simulink library "outp"  (R2021b)
(part 5 of 8)

  VBCM_MirrorFlodPos_flg_Inproc : FVT_lib/outp/OverrideAndLimit  SystemSampleTime=-1  VariantActivationTime=update diagram  Latency=0  AutoFrameSizeCalculation=off
      link override Signal_Limit/_maxval: Value=KOUTP_MirrorFlodPos_flg_maxval
      link override Signal_Limit/_minval: Value=KOUTP_MirrorFlodPos_flg_minval
      link override Signal_Override/_ovrdflg: Value=KOUTP_MirrorFlodPos_flg_ovrdflg
      link override Signal_Override/_ovrdval: Value=KOUTP_MirrorFlodPos_flg_ovrdval
  VBCM_OutMode_enum_Inproc : FVT_lib/outp/OverrideAndLimit  SystemSampleTime=-1  VariantActivationTime=update diagram  Latency=0  AutoFrameSizeCalculation=off
      link override Signal_Limit/_maxval: Value=KOUTP_OutMode_enum_maxval
      link override Signal_Limit/_minval: Value=KOUTP_OutMode_enum_minval
      link override Signal_Override/_ovrdflg: Value=KOUTP_OutMode_enum_ovrdflg
      link override Signal_Override/_ovrdval: Value=KOUTP_OutMode_enum_ovrdval
  VBCM_PTGInnerSW2_enum_Inproc : FVT_lib/outp/OverrideAndLimit  SystemSampleTime=-1  VariantActivationTime=update diagram  Latency=0  AutoFrameSizeCalculation=off
      link override Signal_Limit/_maxval: Value=KOUTP_PTGInnerSW2_enum_maxval
      link override Signal_Limit/_minval: Value=KOUTP_PTGInnerSW2_enum_minval
      link override Signal_Override/_ovrdflg: Value=KOUTP_PTGInnerSW2_enum_ovrdflg
      link override Signal_Override/_ovrdval: Value=KOUTP_PTGInnerSW2_enum_ovrdval
  VBCM_PosLamp_flg_Inproc : FVT_lib/outp/OverrideAndLimit  SystemSampleTime=-1  VariantActivationTime=update diagram  Latency=0  AutoFrameSizeCalculation=off
      link override Signal_Limit/_maxval: Value=KOUTP_PosLamp_flg_maxval
      link override Signal_Limit/_minval: Value=KOUTP_PosLamp_flg_minval
      link override Signal_Override/_ovrdflg: Value=KOUTP_PosLamp_flg_ovrdflg
      link override Signal_Override/_ovrdval: Value=KOUTP_PosLamp_flg_ovrdval
  VBCM_PsDoorSW_flg_Inproc : FVT_lib/outp/OverrideAndLimit  SystemSampleTime=-1  VariantActivationTime=update diagram  Latency=0  AutoFrameSizeCalculation=off
      link override Signal_Limit/_maxval: Value=KOUTP_PsDoorSW_flg_maxval
      link override Signal_Limit/_minval: Value=KOUTP_PsDoorSW_flg_minval
      link override Signal_Override/_ovrdflg: Value=KOUTP_PsDoorSW_flg_ovrdflg
      link override Signal_Override/_ovrdval: Value=KOUTP_PsDoorSW_flg_ovrdval
  VBCM_RBSD_flg_Inproc : FVT_lib/outp/OverrideAndLimit  SystemSampleTime=-1  VariantActivationTime=update diagram  Latency=0  AutoFrameSizeCalculation=off
      link override Signal_Limit/_maxval: Value=KOUTP_RBSD_flg_maxval
      link override Signal_Limit/_minval: Value=KOUTP_RBSD_flg_minval
      link override Signal_Override/_ovrdflg: Value=KOUTP_RBSD_flg_ovrdflg
      link override Signal_Override/_ovrdval: Value=KOUTP_RBSD_flg_ovrdval
  VBCM_RDRL_flg_Inproc : FVT_lib/outp/OverrideAndLimit  SystemSampleTime=-1  VariantActivationTime=update diagram  Latency=0  AutoFrameSizeCalculation=off
      link override Signal_Limit/_maxval: Value=KOUTP_RDRL_flg_maxval
      link override Signal_Limit/_minval: Value=KOUTP_RDRL_flg_minval
      link override Signal_Override/_ovrdflg: Value=KOUTP_RDRL_flg_ovrdflg
      link override Signal_Override/_ovrdval: Value=KOUTP_RDRL_flg_ovrdval
  VBCM_RLDoorSW_flg_Inproc : FVT_lib/outp/OverrideAndLimit  SystemSampleTime=-1  VariantActivationTime=update diagram  Latency=0  AutoFrameSizeCalculation=off
      link override Signal_Limit/_maxval: Value=KOUTP_RLDoorSW_flg_maxval
      link override Signal_Limit/_minval: Value=KOUTP_RLDoorSW_flg_minval
      link override Signal_Override/_ovrdflg: Value=KOUTP_RLDoorSW_flg_ovrdflg
      link override Signal_Override/_ovrdval: Value=KOUTP_RLDoorSW_flg_ovrdval
  VBCM_RRDoorSW_flg_Inproc : FVT_lib/outp/OverrideAndLimit  SystemSampleTime=-1  VariantActivationTime=update diagram  Latency=0  AutoFrameSizeCalculation=off
      link override Signal_Limit/_maxval: Value=KOUTP_RRDoorSW_flg_maxval
      link override Signal_Limit/_minval: Value=KOUTP_RRDoorSW_flg_minval
      link override Signal_Override/_ovrdflg: Value=KOUTP_RRDoorSW_flg_ovrdflg
      link override Signal_Override/_ovrdval: Value=KOUTP_RRDoorSW_flg_ovrdval
  VBCM_RTurnLP_flg_Inproc : FVT_lib/outp/OverrideAndLimit  SystemSampleTime=-1  VariantActivationTime=update diagram  Latency=0  AutoFrameSizeCalculation=off
      link override Signal_Limit/_maxval: Value=KOUTP_RTurnLP_flg_maxval
      link override Signal_Limit/_minval: Value=KOUTP_RTurnLP_flg_minval
      link override Signal_Override/_ovrdflg: Value=KOUTP_RTurnLP_flg_ovrdflg
      link override Signal_Override/_ovrdval: Value=KOUTP_RTurnLP_flg_ovrdval
  VBCM_ReverseLamp_flg_Inproc : FVT_lib/outp/OverrideAndLimit  SystemSampleTime=-1  VariantActivationTime=update diagram  Latency=0  AutoFrameSizeCalculation=off
      link override Signal_Limit/_maxval: Value=KOUTP_ReverseLamp_flg_maxval
      link override Signal_Limit/_minval: Value=KOUTP_ReverseLamp_flg_minval
      link override Signal_Override/_ovrdflg: Value=KOUTP_ReverseLamp_flg_ovrdflg
      link override Signal_Override/_ovrdval: Value=KOUTP_ReverseLamp_flg_ovrdval
  VBCM_RoomLampH_flg_Inproc : FVT_lib/outp/OverrideAndLimit  SystemSampleTime=-1  VariantActivationTime=update diagram  Latency=0  AutoFrameSizeCalculation=off
      link override Signal_Limit/_maxval: Value=KOUTP_RoomLampH_flg_maxval
      link override Signal_Limit/_minval: Value=KOUTP_RoomLampH_flg_minval
      link override Signal_Override/_ovrdflg: Value=KOUTP_RoomLampH_flg_ovrdflg
      link override Signal_Override/_ovrdval: Value=KOUTP_RoomLampH_flg_ovrdval
  VBCM_RoomLampL_flg_Inproc : FVT_lib/outp/OverrideAndLimit  SystemSampleTime=-1  VariantActivationTime=update diagram  Latency=0  AutoFrameSizeCalculation=off
      link override Signal_Limit/_maxval: Value=KOUTP_RoomLampL_flg_maxval
      link override Signal_Limit/_minval: Value=KOUTP_RoomLampL_flg_minval
      link override Signal_Override/_ovrdflg: Value=KOUTP_RoomLampL_flg_ovrdflg
      link override Signal_Override/_ovrdval: Value=KOUTP_RoomLampL_flg_ovrdval
  VBCM_RoomLampMode_flg_Inproc : FVT_lib/outp/OverrideAndLimit  SystemSampleTime=-1  VariantActivationTime=update diagram  Latency=0  AutoFrameSizeCalculation=off
      link override Signal_Limit/_maxval: Value=KOUTP_RoomLampMode_flg_maxval
      link override Signal_Limit/_minval: Value=KOUTP_RoomLampMode_flg_minval
      link override Signal_Override/_ovrdflg: Value=KOUTP_RoomLampMode_flg_ovrdflg
      link override Signal_Override/_ovrdval: Value=KOUTP_RoomLampMode_flg_ovrdval
  VBCM_RrChargingDoorCtrl_enum_Inproc : FVT_lib/outp/OverrideAndLimit  SystemSampleTime=-1  VariantActivationTime=update diagram  Latency=0  AutoFrameSizeCalculation=off
      link override Signal_Limit/_maxval: Value=KOUTP_RrChargingDoorCtrl_enum_maxval
      link override Signal_Limit/_minval: Value=KOUTP_RrChargingDoorCtrl_enum_minval
      link override Signal_Override/_ovrdflg: Value=KOUTP_RrChargingDoorCtrl_enum_ovrdflg
      link override Signal_Override/_ovrdval: Value=KOUTP_RrChargingDoorCtrl_enum_ovrdval
  VBCM_RrDefog_flg_Inproc : FVT_lib/outp/OverrideAndLimit  SystemSampleTime=-1  VariantActivationTime=update diagram  Latency=0  AutoFrameSizeCalculation=off
      link override Signal_Limit/_maxval: Value=KOUTP_RrDefog_flg_maxval
      link override Signal_Limit/_minval: Value=KOUTP_RrDefog_flg_minval
      link override Signal_Override/_ovrdflg: Value=KOUTP_RrDefog_flg_ovrdflg
      link override Signal_Override/_ovrdval: Value=KOUTP_RrDefog_flg_ovrdval
  VBCM_RrFogLamp_flg_Inproc : FVT_lib/outp/OverrideAndLimit  SystemSampleTime=-1  VariantActivationTime=update diagram  Latency=0  AutoFrameSizeCalculation=off
      link override Signal_Limit/_maxval: Value=KOUTP_RrFogLamp_flg_maxval
      link override Signal_Limit/_minval: Value=KOUTP_RrFogLamp_flg_minval
      link override Signal_Override/_ovrdflg: Value=KOUTP_RrFogLamp_flg_ovrdflg
      link override Signal_Override/_ovrdval: Value=KOUTP_RrFogLamp_flg_ovrdval
  VBCM_RrWiper_flg_Inproc : FVT_lib/outp/OverrideAndLimit  SystemSampleTime=-1  VariantActivationTime=update diagram  Latency=0  AutoFrameSizeCalculation=off
      link override Signal_Limit/_maxval: Value=KOUTP_RrWiper_flg_maxval
      link override Signal_Limit/_minval: Value=KOUTP_RrWiper_flg_minval
      link override Signal_Override/_ovrdflg: Value=KOUTP_RrWiper_flg_ovrdflg
      link override Signal_Override/_ovrdval: Value=KOUTP_RrWiper_flg_ovrdval
  VBCM_SPTGDet_flg_Inproc : FVT_lib/outp/OverrideAndLimit  SystemSampleTime=-1  VariantActivationTime=update diagram  Latency=0  AutoFrameSizeCalculation=off
      link override Signal_Limit/_maxval: Value=KOUTP_SPTGDet_flg_maxval
      link override Signal_Limit/_minval: Value=KOUTP_SPTGDet_flg_minval
      link override Signal_Override/_ovrdflg: Value=KOUTP_SPTGDet_flg_ovrdflg
      link override Signal_Override/_ovrdval: Value=KOUTP_SPTGDet_flg_ovrdval
  VBCM_TailgateHDSW_flg_Inproc : FVT_lib/outp/OverrideAndLimit  SystemSampleTime=-1  VariantActivationTime=update diagram  Latency=0  AutoFrameSizeCalculation=off
      link override Signal_Limit/_maxval: Value=KOUTP_TailgateHDSW_flg_maxval
      link override Signal_Limit/_minval: Value=KOUTP_TailgateHDSW_flg_minval
      link override Signal_Override/_ovrdflg: Value=KOUTP_TailgateHDSW_flg_ovrdflg
      link override Signal_Override/_ovrdval: Value=KOUTP_TailgateHDSW_flg_ovrdval
  VBCM_TailgateRemote_enum_Inproc : FVT_lib/outp/OverrideAndLimit  SystemSampleTime=-1  VariantActivationTime=update diagram  Latency=0  AutoFrameSizeCalculation=off
      link override Signal_Limit/_maxval: Value=KOUTP_TailgateRemote_enum_maxval
      link override Signal_Limit/_minval: Value=KOUTP_TailgateRemote_enum_minval
      link override Signal_Override/_ovrdflg: Value=KOUTP_TailgateRemote_enum_ovrdflg
      link override Signal_Override/_ovrdval: Value=KOUTP_TailgateRemote_enum_ovrdval
  VBCM_TailgateSW_flg_Inproc : FVT_lib/outp/OverrideAndLimit  SystemSampleTime=-1  VariantActivationTime=update diagram  Latency=0  AutoFrameSizeCalculation=off
      link override Signal_Limit/_maxval: Value=KOUTP_TailgateSW_flg_maxval
      link override Signal_Limit/_minval: Value=KOUTP_TailgateSW_flg_minval
      link override Signal_Override/_ovrdflg: Value=KOUTP_TailgateSW_flg_ovrdflg
      link override Signal_Override/_ovrdval: Value=KOUTP_TailgateSW_flg_ovrdval
  VBCM_TrunkRel_flg_Inproc : FVT_lib/outp/OverrideAndLimit  SystemSampleTime=-1  VariantActivationTime=update diagram  Latency=0  AutoFrameSizeCalculation=off
      link override Signal_Limit/_maxval: Value=KOUTP_TrunkRel_flg_maxval
      link override Signal_Limit/_minval: Value=KOUTP_TrunkRel_flg_minval
      link override Signal_Override/_ovrdflg: Value=KOUTP_TrunkRel_flg_ovrdflg
      link override Signal_Override/_ovrdval: Value=KOUTP_TrunkRel_flg_ovrdval
  VBCM_User1AmbLightColor_enum_Inproc : FVT_lib/outp/OverrideAndLimit  SystemSampleTime=-1  VariantActivationTime=update diagram  Latency=0  AutoFrameSizeCalculation=off
      link override Signal_Limit/_maxval: Value=KOUTP_User1AmbLightColor_enum_maxval
      link override Signal_Limit/_minval: Value=KOUTP_User1AmbLightColor_enum_minval
      link override Signal_Override/_ovrdflg: Value=KOUTP_User1AmbLightColor_enum_ovrdflg
      link override Signal_Override/_ovrdval: Value=KOUTP_User1AmbLightColor_enum_ovrdval
  VBCM_User1DrAmbLightBrightness_enum_Inproc : FVT_lib/outp/OverrideAndLimit  SystemSampleTime=-1  VariantActivationTime=update diagram  Latency=0  AutoFrameSizeCalculation=off
      link override Signal_Limit/_maxval: Value=KOUTP_User1DrAmbLightBrightness_enum_maxval
      link override Signal_Limit/_minval: Value=KOUTP_User1DrAmbLightBrightness_enum_minval
      link override Signal_Override/_ovrdflg: Value=KOUTP_User1DrAmbLightBrightness_enum_ovrdflg
      link override Signal_Override/_ovrdval: Value=KOUTP_User1DrAmbLightBrightness_enum_ovrdval
  VBCM_User1IPAmbLightBrightness_enum_Inproc : FVT_lib/outp/OverrideAndLimit  SystemSampleTime=-1  VariantActivationTime=update diagram  Latency=0  AutoFrameSizeCalculation=off
      link override Signal_Limit/_maxval: Value=KOUTP_User1IPAmbLightBrightness_enum_maxval
      link override Signal_Limit/_minval: Value=KOUTP_User1IPAmbLightBrightness_enum_minval
      link override Signal_Override/_ovrdflg: Value=KOUTP_User1IPAmbLightBrightness_enum_ovrdflg
      link override Signal_Override/_ovrdval: Value=KOUTP_User1IPAmbLightBrightness_enum_ovrdval
  VBCM_User2AmbLightColor_enum_Inproc : FVT_lib/outp/OverrideAndLimit  SystemSampleTime=-1  VariantActivationTime=update diagram  Latency=0  AutoFrameSizeCalculation=off
      link override Signal_Limit/_maxval: Value=KOUTP_User2AmbLightColor_enum_maxval
      link override Signal_Limit/_minval: Value=KOUTP_User2AmbLightColor_enum_minval
      link override Signal_Override/_ovrdflg: Value=KOUTP_User2AmbLightColor_enum_ovrdflg
      link override Signal_Override/_ovrdval: Value=KOUTP_User2AmbLightColor_enum_ovrdval
  VBCM_User2DrAmbLightBrightness_enum_Inproc : FVT_lib/outp/OverrideAndLimit  SystemSampleTime=-1  VariantActivationTime=update diagram  Latency=0  AutoFrameSizeCalculation=off
      link override Signal_Limit/_maxval: Value=KOUTP_User2DrAmbLightBrightness_enum_maxval
      link override Signal_Limit/_minval: Value=KOUTP_User2DrAmbLightBrightness_enum_minval
      link override Signal_Override/_ovrdflg: Value=KOUTP_User2DrAmbLightBrightness_enum_ovrdflg
      link override Signal_Override/_ovrdval: Value=KOUTP_User2DrAmbLightBrightness_enum_ovrdval
  VBCM_User2IPAmbLightBrightness_enum_Inproc : FVT_lib/outp/OverrideAndLimit  SystemSampleTime=-1  VariantActivationTime=update diagram  Latency=0  AutoFrameSizeCalculation=off
      link override Signal_Limit/_maxval: Value=KOUTP_User2IPAmbLightBrightness_enum_maxval
      link override Signal_Limit/_minval: Value=KOUTP_User2IPAmbLightBrightness_enum_minval
      link override Signal_Override/_ovrdflg: Value=KOUTP_User2IPAmbLightBrightness_enum_ovrdflg
      link override Signal_Override/_ovrdval: Value=KOUTP_User2IPAmbLightBrightness_enum_ovrdval
  VBCM_User3AmbLightColor_enum_Inproc : FVT_lib/outp/OverrideAndLimit  SystemSampleTime=-1  VariantActivationTime=update diagram  Latency=0  AutoFrameSizeCalculation=off
      link override Signal_Limit/_maxval: Value=KOUTP_User3AmbLightColor_enum_maxval
      link override Signal_Limit/_minval: Value=KOUTP_User3AmbLightColor_enum_minval
      link override Signal_Override/_ovrdflg: Value=KOUTP_User3AmbLightColor_enum_ovrdflg
      link override Signal_Override/_ovrdval: Value=KOUTP_User3AmbLightColor_enum_ovrdval
  VBCM_User3DrAmbLightBrightness_enum_Inproc : FVT_lib/outp/OverrideAndLimit  SystemSampleTime=-1  VariantActivationTime=update diagram  Latency=0  AutoFrameSizeCalculation=off
      link override Signal_Limit/_maxval: Value=KOUTP_User3DrAmbLightBrightness_enum_maxval
      link override Signal_Limit/_minval: Value=KOUTP_User3DrAmbLightBrightness_enum_minval
      link override Signal_Override/_ovrdflg: Value=KOUTP_User3DrAmbLightBrightness_enum_ovrdflg
      link override Signal_Override/_ovrdval: Value=KOUTP_User3DrAmbLightBrightness_enum_ovrdval
  VBCM_User3IPAmbLightBrightness_enum_Inproc : FVT_lib/outp/OverrideAndLimit  SystemSampleTime=-1  VariantActivationTime=update diagram  Latency=0  AutoFrameSizeCalculation=off
      link override Signal_Limit/_maxval: Value=KOUTP_User3IPAmbLightBrightness_enum_maxval
      link override Signal_Limit/_minval: Value=KOUTP_User3IPAmbLightBrightness_enum_minval
      link override Signal_Override/_ovrdflg: Value=KOUTP_User3IPAmbLightBrightness_enum_ovrdflg
      link override Signal_Override/_ovrdval: Value=KOUTP_User3IPAmbLightBrightness_enum_ovrdval
  VBCM_User4AmbLightColor_enum_Inproc : FVT_lib/outp/OverrideAndLimit  SystemSampleTime=-1  VariantActivationTime=update diagram  Latency=0  AutoFrameSizeCalculation=off
      link override Signal_Limit/_maxval: Value=KOUTP_User4AmbLightColor_enum_maxval
      link override Signal_Limit/_minval: Value=KOUTP_User4AmbLightColor_enum_minval
      link override Signal_Override/_ovrdflg: Value=KOUTP_User4AmbLightColor_enum_ovrdflg
      link override Signal_Override/_ovrdval: Value=KOUTP_User4AmbLightColor_enum_ovrdval
  VBCM_User4DrAmbLightBrightness_enum_Inproc : FVT_lib/outp/OverrideAndLimit  SystemSampleTime=-1  VariantActivationTime=update diagram  Latency=0  AutoFrameSizeCalculation=off
      link override Signal_Limit/_maxval: Value=KOUTP_User4DrAmbLightBrightness_enum_maxval
      link override Signal_Limit/_minval: Value=KOUTP_User4DrAmbLightBrightness_enum_minval
      link override Signal_Override/_ovrdflg: Value=KOUTP_User4DrAmbLightBrightness_enum_ovrdflg
      link override Signal_Override/_ovrdval: Value=KOUTP_User4DrAmbLightBrightness_enum_ovrdval
  VBCM_User4IPAmbLightBrightness_enum_Inproc : FVT_lib/outp/OverrideAndLimit  SystemSampleTime=-1  VariantActivationTime=update diagram  Latency=0  AutoFrameSizeCalculation=off
      link override Signal_Limit/_maxval: Value=KOUTP_User4IPAmbLightBrightness_enum_maxval
      link override Signal_Limit/_minval: Value=KOUTP_User4IPAmbLightBrightness_enum_minval
      link override Signal_Override/_ovrdflg: Value=KOUTP_User4IPAmbLightBrightness_enum_ovrdflg
      link override Signal_Override/_ovrdval: Value=KOUTP_User4IPAmbLightBrightness_enum_ovrdval
  VBCM_User5AmbLightColor_enum_Inproc : FVT_lib/outp/OverrideAndLimit  SystemSampleTime=-1  VariantActivationTime=update diagram  Latency=0  AutoFrameSizeCalculation=off
      link override Signal_Limit/_maxval: Value=KOUTP_User5AmbLightColor_enum_maxval
      link override Signal_Limit/_minval: Value=KOUTP_User5AmbLightColor_enum_minval
      link override Signal_Override/_ovrdflg: Value=KOUTP_User5AmbLightColor_enum_ovrdflg
      link override Signal_Override/_ovrdval: Value=KOUTP_User5AmbLightColor_enum_ovrdval
  VBCM_User5DrAmbLightBrightness_enum_Inproc : FVT_lib/outp/OverrideAndLimit  SystemSampleTime=-1  VariantActivationTime=update diagram  Latency=0  AutoFrameSizeCalculation=off
      link override Signal_Limit/_maxval: Value=KOUTP_User5DrAmbLightBrightness_enum_maxval
      link override Signal_Limit/_minval: Value=KOUTP_User5DrAmbLightBrightness_enum_minval
      link override Signal_Override/_ovrdflg: Value=KOUTP_User5DrAmbLightBrightness_enum_ovrdflg
      link override Signal_Override/_ovrdval: Value=KOUTP_User5DrAmbLightBrightness_enum_ovrdval
  VBCM_User5IPAmbLightBrightness_enum_Inproc : FVT_lib/outp/OverrideAndLimit  SystemSampleTime=-1  VariantActivationTime=update diagram  Latency=0  AutoFrameSizeCalculation=off
      link override Signal_Limit/_maxval: Value=KOUTP_User5IPAmbLightBrightness_enum_maxval
      link override Signal_Limit/_minval: Value=KOUTP_User5IPAmbLightBrightness_enum_minval
      link override Signal_Override/_ovrdflg: Value=KOUTP_User5IPAmbLightBrightness_enum_ovrdflg
      link override Signal_Override/_ovrdval: Value=KOUTP_User5IPAmbLightBrightness_enum_ovrdval
  VBCM_User6AmbLightColor_enum_Inproc : FVT_lib/outp/OverrideAndLimit  SystemSampleTime=-1  VariantActivationTime=update diagram  Latency=0  AutoFrameSizeCalculation=off
      link override Signal_Limit/_maxval: Value=KOUTP_User6AmbLightColor_enum_maxval
      link override Signal_Limit/_minval: Value=KOUTP_User6AmbLightColor_enum_minval
      link override Signal_Override/_ovrdflg: Value=KOUTP_User6AmbLightColor_enum_ovrdflg
      link override Signal_Override/_ovrdval: Value=KOUTP_User6AmbLightColor_enum_ovrdval
  VBCM_User6DrAmbLightBrightness_enum_Inproc : FVT_lib/outp/OverrideAndLimit  SystemSampleTime=-1  VariantActivationTime=update diagram  Latency=0  AutoFrameSizeCalculation=off
      link override Signal_Limit/_maxval: Value=KOUTP_User6DrAmbLightBrightness_enum_maxval
      link override Signal_Limit/_minval: Value=KOUTP_User6DrAmbLightBrightness_enum_minval
      link override Signal_Override/_ovrdflg: Value=KOUTP_User6DrAmbLightBrightness_enum_ovrdflg
      link override Signal_Override/_ovrdval: Value=KOUTP_User6DrAmbLightBrightness_enum_ovrdval
  VBCM_User6IPAmbLightBrightness_enum_Inproc : FVT_lib/outp/OverrideAndLimit  SystemSampleTime=-1  VariantActivationTime=update diagram  Latency=0  AutoFrameSizeCalculation=off
      link override Signal_Limit/_maxval: Value=KOUTP_User6IPAmbLightBrightness_enum_maxval
      link override Signal_Limit/_minval: Value=KOUTP_User6IPAmbLightBrightness_enum_minval
      link override Signal_Override/_ovrdflg: Value=KOUTP_User6IPAmbLightBrightness_enum_ovrdflg
      link override Signal_Override/_ovrdval: Value=KOUTP_User6IPAmbLightBrightness_enum_ovrdval
  VBCM_WasherCtrl_enum_Inproc : FVT_lib/outp/OverrideAndLimit  SystemSampleTime=-1  VariantActivationTime=update diagram  Latency=0  AutoFrameSizeCalculation=off
      link override Signal_Limit/_maxval: Value=KOUTP_WasherCtrl_enum_maxval
      link override Signal_Limit/_minval: Value=KOUTP_WasherCtrl_enum_minval
      link override Signal_Override/_ovrdflg: Value=KOUTP_WasherCtrl_enum_ovrdflg
      link override Signal_Override/_ovrdval: Value=KOUTP_WasherCtrl_enum_ovrdval
  VBCM_WiperFixMode_flg_Inproc : FVT_lib/outp/OverrideAndLimit  SystemSampleTime=-1  VariantActivationTime=update diagram  Latency=0  AutoFrameSizeCalculation=off
      link override Signal_Limit/_maxval: Value=KOUTP_WiperFixMode_flg_maxval
      link override Signal_Limit/_minval: Value=KOUTP_WiperFixMode_flg_minval
      link override Signal_Override/_ovrdflg: Value=KOUTP_WiperFixMode_flg_ovrdflg
      link override Signal_Override/_ovrdval: Value=KOUTP_WiperFixMode_flg_ovrdval
  VBCM_fUnlockSingle_flg_Inproc : FVT_lib/outp/OverrideAndLimit  SystemSampleTime=-1  VariantActivationTime=update diagram  Latency=0  AutoFrameSizeCalculation=off
      link override Signal_Limit/_maxval: Value=KOUTP_fUnlockSingle_flg_maxval
      link override Signal_Limit/_minval: Value=KOUTP_fUnlockSingle_flg_minval
      link override Signal_Override/_ovrdflg: Value=KOUTP_fUnlockSingle_flg_ovrdflg
      link override Signal_Override/_ovrdval: Value=KOUTP_fUnlockSingle_flg_ovrdval
  VDDM_5vAPS1PwrErrDTC_raw32_Inproc : FVT_lib/outp/OverrideAndLimit  SystemSampleTime=-1  VariantActivationTime=update diagram  Latency=0  AutoFrameSizeCalculation=off
      link override Signal_Limit/_maxval: Value=KOUTP_5vAPS1PwrErrDTC_raw32_maxval
      link override Signal_Limit/_minval: Value=KOUTP_5vAPS1PwrErrDTC_raw32_minval
      link override Signal_Override/_ovrdflg: Value=KOUTP_5vAPS1PwrErrDTC_raw32_ovrdflg
      link override Signal_Override/_ovrdval: Value=KOUTP_5vAPS1PwrErrDTC_raw32_ovrdval
  VDDM_5vAPS2PwrErrDTC_raw32_Inproc : FVT_lib/outp/OverrideAndLimit  SystemSampleTime=-1  VariantActivationTime=update diagram  Latency=0  AutoFrameSizeCalculation=off
      link override Signal_Limit/_maxval: Value=KOUTP_5vAPS2PwrErrDTC_raw32_maxval
      link override Signal_Limit/_minval: Value=KOUTP_5vAPS2PwrErrDTC_raw32_minval
      link override Signal_Override/_ovrdflg: Value=KOUTP_5vAPS2PwrErrDTC_raw32_ovrdflg
      link override Signal_Override/_ovrdval: Value=KOUTP_5vAPS2PwrErrDTC_raw32_ovrdval
  VDDM_ACCAccelCmdErrDetDTC_raw32_Inproc : FVT_lib/outp/OverrideAndLimit  SystemSampleTime=-1  VariantActivationTime=update diagram  Latency=0  AutoFrameSizeCalculation=off
      link override Signal_Limit/_maxval: Value=KOUTP_ACCAccelCmdErrDetDTC_raw32_maxval
      link override Signal_Limit/_minval: Value=KOUTP_ACCAccelCmdErrDetDTC_raw32_minval
      link override Signal_Override/_ovrdflg: Value=KOUTP_ACCAccelCmdErrDetDTC_raw32_ovrdflg
      link override Signal_Override/_ovrdval: Value=KOUTP_ACCAccelCmdErrDetDTC_raw32_ovrdval
  VDDM_ACCMalfuncDetDTC_raw32_Inproc : FVT_lib/outp/OverrideAndLimit  SystemSampleTime=-1  VariantActivationTime=update diagram  Latency=0  AutoFrameSizeCalculation=off
      link override Signal_Limit/_maxval: Value=KOUTP_ACCMalfuncDetDTC_raw32_maxval
      link override Signal_Limit/_minval: Value=KOUTP_ACCMalfuncDetDTC_raw32_minval
      link override Signal_Override/_ovrdflg: Value=KOUTP_ACCMalfuncDetDTC_raw32_ovrdflg
      link override Signal_Override/_ovrdval: Value=KOUTP_ACCMalfuncDetDTC_raw32_ovrdval
  VDDM_APS1SigOoRDTC_raw32_Inproc : FVT_lib/outp/OverrideAndLimit  SystemSampleTime=-1  VariantActivationTime=update diagram  Latency=0  AutoFrameSizeCalculation=off
      link override Signal_Limit/_maxval: Value=KOUTP_APS1SigOoRDTC_raw32_maxval
      link override Signal_Limit/_minval: Value=KOUTP_APS1SigOoRDTC_raw32_minval
      link override Signal_Override/_ovrdflg: Value=KOUTP_APS1SigOoRDTC_raw32_ovrdflg
      link override Signal_Override/_ovrdval: Value=KOUTP_APS1SigOoRDTC_raw32_ovrdval
  VDDM_APS2SigOoRDTC_raw32_Inproc : FVT_lib/outp/OverrideAndLimit  SystemSampleTime=-1  VariantActivationTime=update diagram  Latency=0  AutoFrameSizeCalculation=off
      link override Signal_Limit/_maxval: Value=KOUTP_APS2SigOoRDTC_raw32_maxval
      link override Signal_Limit/_minval: Value=KOUTP_APS2SigOoRDTC_raw32_minval
      link override Signal_Override/_ovrdflg: Value=KOUTP_APS2SigOoRDTC_raw32_ovrdflg
      link override Signal_Override/_ovrdval: Value=KOUTP_APS2SigOoRDTC_raw32_ovrdval
  VDDM_APSCorrErrDTC_raw32_Inproc : FVT_lib/outp/OverrideAndLimit  SystemSampleTime=-1  VariantActivationTime=update diagram  Latency=0  AutoFrameSizeCalculation=off
      link override Signal_Limit/_maxval: Value=KOUTP_APSCorrErrDTC_raw32_maxval
      link override Signal_Limit/_minval: Value=KOUTP_APSCorrErrDTC_raw32_minval
      link override Signal_Override/_ovrdflg: Value=KOUTP_APSCorrErrDTC_raw32_ovrdflg
      link override Signal_Override/_ovrdval: Value=KOUTP_APSCorrErrDTC_raw32_ovrdval
  VDDM_BMSRdyDTC_raw32_Inproc : FVT_lib/outp/OverrideAndLimit  SystemSampleTime=-1  VariantActivationTime=update diagram  Latency=0  AutoFrameSizeCalculation=off
      link override Signal_Limit/_maxval: Value=KOUTP_BMSRdyDTC_raw32_maxval
      link override Signal_Limit/_minval: Value=KOUTP_BMSRdyDTC_raw32_minval
      link override Signal_Override/_ovrdflg: Value=KOUTP_BMSRdyDTC_raw32_ovrdflg
      link override Signal_Override/_ovrdval: Value=KOUTP_BMSRdyDTC_raw32_ovrdval
  VDDM_BMSSigErrDetDTC_raw32_Inproc : FVT_lib/outp/OverrideAndLimit  SystemSampleTime=-1  VariantActivationTime=update diagram  Latency=0  AutoFrameSizeCalculation=off
      link override Signal_Limit/_maxval: Value=KOUTP_BMSSigErrDetDTC_raw32_maxval
      link override Signal_Limit/_minval: Value=KOUTP_BMSSigErrDetDTC_raw32_minval
      link override Signal_Override/_ovrdflg: Value=KOUTP_BMSSigErrDetDTC_raw32_ovrdflg
      link override Signal_Override/_ovrdval: Value=KOUTP_BMSSigErrDetDTC_raw32_ovrdval
  VDDM_BrkSWErrDTC_raw32_Inproc : FVT_lib/outp/OverrideAndLimit  SystemSampleTime=-1  VariantActivationTime=update diagram  Latency=0  AutoFrameSizeCalculation=off
      link override Signal_Limit/_maxval: Value=KOUTP_BrkSWErrDTC_raw32_maxval
      link override Signal_Limit/_minval: Value=KOUTP_BrkSWErrDTC_raw32_minval
      link override Signal_Override/_ovrdflg: Value=KOUTP_BrkSWErrDTC_raw32_ovrdflg
      link override Signal_Override/_ovrdval: Value=KOUTP_BrkSWErrDTC_raw32_ovrdval
  VDDM_BrkSWNoBacDTC_raw32_Inproc : FVT_lib/outp/OverrideAndLimit  SystemSampleTime=-1  VariantActivationTime=update diagram  Latency=0  AutoFrameSizeCalculation=off
      link override Signal_Limit/_maxval: Value=KOUTP_BrkSWNoBacDTC_raw32_maxval
      link override Signal_Limit/_minval: Value=KOUTP_BrkSWNoBacDTC_raw32_minval
      link override Signal_Override/_ovrdflg: Value=KOUTP_BrkSWNoBacDTC_raw32_ovrdflg
      link override Signal_Override/_ovrdval: Value=KOUTP_BrkSWNoBacDTC_raw32_ovrdval
  VDDM_C1ABM1CSDTC_raw32_Inproc : FVT_lib/outp/OverrideAndLimit  SystemSampleTime=-1  VariantActivationTime=update diagram  Latency=0  AutoFrameSizeCalculation=off
      link override Signal_Limit/_maxval: Value=KOUTP_C1ABM1CSDTC_raw32_maxval
      link override Signal_Limit/_minval: Value=KOUTP_C1ABM1CSDTC_raw32_minval
      link override Signal_Override/_ovrdflg: Value=KOUTP_C1ABM1CSDTC_raw32_ovrdflg
      link override Signal_Override/_ovrdval: Value=KOUTP_C1ABM1CSDTC_raw32_ovrdval
  VDDM_C1ABM1LCDTC_raw32_Inproc : FVT_lib/outp/OverrideAndLimit  SystemSampleTime=-1  VariantActivationTime=update diagram  Latency=0  AutoFrameSizeCalculation=off
      link override Signal_Limit/_maxval: Value=KOUTP_C1ABM1LCDTC_raw32_maxval
      link override Signal_Limit/_minval: Value=KOUTP_C1ABM1LCDTC_raw32_minval
      link override Signal_Override/_ovrdflg: Value=KOUTP_C1ABM1LCDTC_raw32_ovrdflg
      link override Signal_Override/_ovrdval: Value=KOUTP_C1ABM1LCDTC_raw32_ovrdval
  VDDM_C1ABM1RCDTC_raw32_Inproc : FVT_lib/outp/OverrideAndLimit  SystemSampleTime=-1  VariantActivationTime=update diagram  Latency=0  AutoFrameSizeCalculation=off
      link override Signal_Limit/_maxval: Value=KOUTP_C1ABM1RCDTC_raw32_maxval
      link override Signal_Limit/_minval: Value=KOUTP_C1ABM1RCDTC_raw32_minval
      link override Signal_Override/_ovrdflg: Value=KOUTP_C1ABM1RCDTC_raw32_ovrdflg
      link override Signal_Override/_ovrdval: Value=KOUTP_C1ABM1RCDTC_raw32_ovrdval
  VDDM_C1EPAS2LCDTC_raw32_Inproc : FVT_lib/outp/OverrideAndLimit  SystemSampleTime=-1  VariantActivationTime=update diagram  Latency=0  AutoFrameSizeCalculation=off
      link override Signal_Limit/_maxval: Value=KOUTP_C1EPAS2LCDTC_raw32_maxval
      link override Signal_Limit/_minval: Value=KOUTP_C1EPAS2LCDTC_raw32_minval
      link override Signal_Override/_ovrdflg: Value=KOUTP_C1EPAS2LCDTC_raw32_ovrdflg
      link override Signal_Override/_ovrdval: Value=KOUTP_C1EPAS2LCDTC_raw32_ovrdval
  VDDM_C3BMS1CSDTC_raw32_Inproc : FVT_lib/outp/OverrideAndLimit  SystemSampleTime=-1  VariantActivationTime=update diagram  Latency=0  AutoFrameSizeCalculation=off
      link override Signal_Limit/_maxval: Value=KOUTP_C3BMS1CSDTC_raw32_maxval
      link override Signal_Limit/_minval: Value=KOUTP_C3BMS1CSDTC_raw32_minval
      link override Signal_Override/_ovrdflg: Value=KOUTP_C3BMS1CSDTC_raw32_ovrdflg
      link override Signal_Override/_ovrdval: Value=KOUTP_C3BMS1CSDTC_raw32_ovrdval
  VDDM_C3BMS1LCDTC_raw32_Inproc : FVT_lib/outp/OverrideAndLimit  SystemSampleTime=-1  VariantActivationTime=update diagram  Latency=0  AutoFrameSizeCalculation=off
      link override Signal_Limit/_maxval: Value=KOUTP_C3BMS1LCDTC_raw32_maxval
      link override Signal_Limit/_minval: Value=KOUTP_C3BMS1LCDTC_raw32_minval
      link override Signal_Override/_ovrdflg: Value=KOUTP_C3BMS1LCDTC_raw32_ovrdflg
      link override Signal_Override/_ovrdval: Value=KOUTP_C3BMS1LCDTC_raw32_ovrdval
  VDDM_C3BMS1RCDTC_raw32_Inproc : FVT_lib/outp/OverrideAndLimit  SystemSampleTime=-1  VariantActivationTime=update diagram  Latency=0  AutoFrameSizeCalculation=off
      link override Signal_Limit/_maxval: Value=KOUTP_C3BMS1RCDTC_raw32_maxval
      link override Signal_Limit/_minval: Value=KOUTP_C3BMS1RCDTC_raw32_minval
      link override Signal_Override/_ovrdflg: Value=KOUTP_C3BMS1RCDTC_raw32_ovrdflg
      link override Signal_Override/_ovrdval: Value=KOUTP_C3BMS1RCDTC_raw32_ovrdval
  VDDM_C3BMS6CSDTC_raw32_Inproc : FVT_lib/outp/OverrideAndLimit  SystemSampleTime=-1  VariantActivationTime=update diagram  Latency=0  AutoFrameSizeCalculation=off
      link override Signal_Limit/_maxval: Value=KOUTP_C3BMS6CSDTC_raw32_maxval
      link override Signal_Limit/_minval: Value=KOUTP_C3BMS6CSDTC_raw32_minval
      link override Signal_Override/_ovrdflg: Value=KOUTP_C3BMS6CSDTC_raw32_ovrdflg
      link override Signal_Override/_ovrdval: Value=KOUTP_C3BMS6CSDTC_raw32_ovrdval
  VDDM_C3BMS6LCDTC_raw32_Inproc : FVT_lib/outp/OverrideAndLimit  SystemSampleTime=-1  VariantActivationTime=update diagram  Latency=0  AutoFrameSizeCalculation=off
      link override Signal_Limit/_maxval: Value=KOUTP_C3BMS6LCDTC_raw32_maxval
      link override Signal_Limit/_minval: Value=KOUTP_C3BMS6LCDTC_raw32_minval
      link override Signal_Override/_ovrdflg: Value=KOUTP_C3BMS6LCDTC_raw32_ovrdflg
      link override Signal_Override/_ovrdval: Value=KOUTP_C3BMS6LCDTC_raw32_ovrdval
  VDDM_C3BMS6RCDTC_raw32_Inproc : FVT_lib/outp/OverrideAndLimit  SystemSampleTime=-1  VariantActivationTime=update diagram  Latency=0  AutoFrameSizeCalculation=off
      link override Signal_Limit/_maxval: Value=KOUTP_C3BMS6RCDTC_raw32_maxval
      link override Signal_Limit/_minval: Value=KOUTP_C3BMS6RCDTC_raw32_minval
      link override Signal_Override/_ovrdflg: Value=KOUTP_C3BMS6RCDTC_raw32_ovrdflg
      link override Signal_Override/_ovrdval: Value=KOUTP_C3BMS6RCDTC_raw32_ovrdval
  VDDM_C3CCU1CSDTC_raw32_Inproc : FVT_lib/outp/OverrideAndLimit  SystemSampleTime=-1  VariantActivationTime=update diagram  Latency=0  AutoFrameSizeCalculation=off
      link override Signal_Limit/_maxval: Value=KOUTP_C3CCU1CSDTC_raw32_maxval
      link override Signal_Limit/_minval: Value=KOUTP_C3CCU1CSDTC_raw32_minval
      link override Signal_Override/_ovrdflg: Value=KOUTP_C3CCU1CSDTC_raw32_ovrdflg
      link override Signal_Override/_ovrdval: Value=KOUTP_C3CCU1CSDTC_raw32_ovrdval
  VDDM_C3CCU1LCDTC_raw32_Inproc : FVT_lib/outp/OverrideAndLimit  SystemSampleTime=-1  VariantActivationTime=update diagram  Latency=0  AutoFrameSizeCalculation=off
      link override Signal_Limit/_maxval: Value=KOUTP_C3CCU1LCDTC_raw32_maxval
      link override Signal_Limit/_minval: Value=KOUTP_C3CCU1LCDTC_raw32_minval
      link override Signal_Override/_ovrdflg: Value=KOUTP_C3CCU1LCDTC_raw32_ovrdflg
      link override Signal_Override/_ovrdval: Value=KOUTP_C3CCU1LCDTC_raw32_ovrdval
  VDDM_C3CCU1RCDTC_raw32_Inproc : FVT_lib/outp/OverrideAndLimit  SystemSampleTime=-1  VariantActivationTime=update diagram  Latency=0  AutoFrameSizeCalculation=off
      link override Signal_Limit/_maxval: Value=KOUTP_C3CCU1RCDTC_raw32_maxval
      link override Signal_Limit/_minval: Value=KOUTP_C3CCU1RCDTC_raw32_minval
      link override Signal_Override/_ovrdflg: Value=KOUTP_C3CCU1RCDTC_raw32_ovrdflg
      link override Signal_Override/_ovrdval: Value=KOUTP_C3CCU1RCDTC_raw32_ovrdval
  VDDM_C3CCU2CSDTC_raw32_Inproc : FVT_lib/outp/OverrideAndLimit  SystemSampleTime=-1  VariantActivationTime=update diagram  Latency=0  AutoFrameSizeCalculation=off
      link override Signal_Limit/_maxval: Value=KOUTP_C3CCU2CSDTC_raw32_maxval
      link override Signal_Limit/_minval: Value=KOUTP_C3CCU2CSDTC_raw32_minval
      link override Signal_Override/_ovrdflg: Value=KOUTP_C3CCU2CSDTC_raw32_ovrdflg
      link override Signal_Override/_ovrdval: Value=KOUTP_C3CCU2CSDTC_raw32_ovrdval
  VDDM_C3CCU2LCDTC_raw32_Inproc : FVT_lib/outp/OverrideAndLimit  SystemSampleTime=-1  VariantActivationTime=update diagram  Latency=0  AutoFrameSizeCalculation=off
      link override Signal_Limit/_maxval: Value=KOUTP_C3CCU2LCDTC_raw32_maxval
      link override Signal_Limit/_minval: Value=KOUTP_C3CCU2LCDTC_raw32_minval
      link override Signal_Override/_ovrdflg: Value=KOUTP_C3CCU2LCDTC_raw32_ovrdflg
      link override Signal_Override/_ovrdval: Value=KOUTP_C3CCU2LCDTC_raw32_ovrdval
  VDDM_C3CCU2RCDTC_raw32_Inproc : FVT_lib/outp/OverrideAndLimit  SystemSampleTime=-1  VariantActivationTime=update diagram  Latency=0  AutoFrameSizeCalculation=off
      link override Signal_Limit/_maxval: Value=KOUTP_C3CCU2RCDTC_raw32_maxval
      link override Signal_Limit/_minval: Value=KOUTP_C3CCU2RCDTC_raw32_minval
      link override Signal_Override/_ovrdflg: Value=KOUTP_C3CCU2RCDTC_raw32_ovrdflg
      link override Signal_Override/_ovrdval: Value=KOUTP_C3CCU2RCDTC_raw32_ovrdval
  VDDM_CCMalfuncDetDTC_raw32_Inproc : FVT_lib/outp/OverrideAndLimit  SystemSampleTime=-1  VariantActivationTime=update diagram  Latency=0  AutoFrameSizeCalculation=off
      link override Signal_Limit/_maxval: Value=KOUTP_CCMalfuncDetDTC_raw32_maxval
      link override Signal_Limit/_minval: Value=KOUTP_CCMalfuncDetDTC_raw32_minval
      link override Signal_Override/_ovrdflg: Value=KOUTP_CCMalfuncDetDTC_raw32_ovrdflg
      link override Signal_Override/_ovrdval: Value=KOUTP_CCMalfuncDetDTC_raw32_ovrdval
  VDDM_CCUSigErrDetDTC_raw32_Inproc : FVT_lib/outp/OverrideAndLimit  SystemSampleTime=-1  VariantActivationTime=update diagram  Latency=0  AutoFrameSizeCalculation=off
      link override Signal_Limit/_maxval: Value=KOUTP_CCUSigErrDetDTC_raw32_maxval
      link override Signal_Limit/_minval: Value=KOUTP_CCUSigErrDetDTC_raw32_minval
      link override Signal_Override/_ovrdflg: Value=KOUTP_CCUSigErrDetDTC_raw32_ovrdflg
      link override Signal_Override/_ovrdval: Value=KOUTP_CCUSigErrDetDTC_raw32_ovrdval
  VDDM_DCDC4PreDTC_raw32_Inproc : FVT_lib/outp/OverrideAndLimit  SystemSampleTime=-1  VariantActivationTime=update diagram  Latency=0  AutoFrameSizeCalculation=off
      link override Signal_Limit/_maxval: Value=KOUTP_DCDC4PreDTC_raw32_maxval
      link override Signal_Limit/_minval: Value=KOUTP_DCDC4PreDTC_raw32_minval
      link override Signal_Override/_ovrdflg: Value=KOUTP_DCDC4PreDTC_raw32_ovrdflg
      link override Signal_Override/_ovrdval: Value=KOUTP_DCDC4PreDTC_raw32_ovrdval
  VDDM_DCDCDisDTC_raw32_Inproc : FVT_lib/outp/OverrideAndLimit  SystemSampleTime=-1  VariantActivationTime=update diagram  Latency=0  AutoFrameSizeCalculation=off
      link override Signal_Limit/_maxval: Value=KOUTP_DCDCDisDTC_raw32_maxval
      link override Signal_Limit/_minval: Value=KOUTP_DCDCDisDTC_raw32_minval
      link override Signal_Override/_ovrdflg: Value=KOUTP_DCDCDisDTC_raw32_ovrdflg
      link override Signal_Override/_ovrdval: Value=KOUTP_DCDCDisDTC_raw32_ovrdval
  VDDM_DCDCEnaDTC_raw32_Inproc : FVT_lib/outp/OverrideAndLimit  SystemSampleTime=-1  VariantActivationTime=update diagram  Latency=0  AutoFrameSizeCalculation=off
      link override Signal_Limit/_maxval: Value=KOUTP_DCDCEnaDTC_raw32_maxval
      link override Signal_Limit/_minval: Value=KOUTP_DCDCEnaDTC_raw32_minval
      link override Signal_Override/_ovrdflg: Value=KOUTP_DCDCEnaDTC_raw32_ovrdflg
      link override Signal_Override/_ovrdval: Value=KOUTP_DCDCEnaDTC_raw32_ovrdval
  VDDM_DiagFLTSDTC_raw32_Inproc : FVT_lib/outp/OverrideAndLimit  SystemSampleTime=-1  VariantActivationTime=update diagram  Latency=0  AutoFrameSizeCalculation=off
      link override Signal_Limit/_maxval: Value=KOUTP_DiagFLTSDTC_raw32_maxval
      link override Signal_Limit/_minval: Value=KOUTP_DiagFLTSDTC_raw32_minval
      link override Signal_Override/_ovrdflg: Value=KOUTP_DiagFLTSDTC_raw32_ovrdflg
      link override Signal_Override/_ovrdval: Value=KOUTP_DiagFLTSDTC_raw32_ovrdval
  VDDM_DiagFRTSDTC_raw32_Inproc : FVT_lib/outp/OverrideAndLimit  SystemSampleTime=-1  VariantActivationTime=update diagram  Latency=0  AutoFrameSizeCalculation=off
      link override Signal_Limit/_maxval: Value=KOUTP_DiagFRTSDTC_raw32_maxval
      link override Signal_Limit/_minval: Value=KOUTP_DiagFRTSDTC_raw32_minval
      link override Signal_Override/_ovrdflg: Value=KOUTP_DiagFRTSDTC_raw32_ovrdflg
      link override Signal_Override/_ovrdval: Value=KOUTP_DiagFRTSDTC_raw32_ovrdval
  VDDM_DiagHCrashDTC_raw32_Inproc : FVT_lib/outp/OverrideAndLimit  SystemSampleTime=-1  VariantActivationTime=update diagram  Latency=0  AutoFrameSizeCalculation=off
      link override Signal_Limit/_maxval: Value=KOUTP_DiagHCrashDTC_raw32_maxval
      link override Signal_Limit/_minval: Value=KOUTP_DiagHCrashDTC_raw32_minval
      link override Signal_Override/_ovrdflg: Value=KOUTP_DiagHCrashDTC_raw32_ovrdflg
      link override Signal_Override/_ovrdval: Value=KOUTP_DiagHCrashDTC_raw32_ovrdval
  VDDM_DiagRLTSDTC_raw32_Inproc : FVT_lib/outp/OverrideAndLimit  SystemSampleTime=-1  VariantActivationTime=update diagram  Latency=0  AutoFrameSizeCalculation=off
      link override Signal_Limit/_maxval: Value=KOUTP_DiagRLTSDTC_raw32_maxval
      link override Signal_Limit/_minval: Value=KOUTP_DiagRLTSDTC_raw32_minval
      link override Signal_Override/_ovrdflg: Value=KOUTP_DiagRLTSDTC_raw32_ovrdflg
      link override Signal_Override/_ovrdval: Value=KOUTP_DiagRLTSDTC_raw32_ovrdval
  VDDM_DiagRRTSDTC_raw32_Inproc : FVT_lib/outp/OverrideAndLimit  SystemSampleTime=-1  VariantActivationTime=update diagram  Latency=0  AutoFrameSizeCalculation=off
      link override Signal_Limit/_maxval: Value=KOUTP_DiagRRTSDTC_raw32_maxval
      link override Signal_Limit/_minval: Value=KOUTP_DiagRRTSDTC_raw32_minval
      link override Signal_Override/_ovrdflg: Value=KOUTP_DiagRRTSDTC_raw32_ovrdflg
      link override Signal_Override/_ovrdval: Value=KOUTP_DiagRRTSDTC_raw32_ovrdval
  VDDM_DrStSWDTC_raw32_Inproc : FVT_lib/outp/OverrideAndLimit  SystemSampleTime=-1  VariantActivationTime=update diagram  Latency=0  AutoFrameSizeCalculation=off
      link override Signal_Limit/_maxval: Value=KOUTP_DrStSWDTC_raw32_maxval
      link override Signal_Limit/_minval: Value=KOUTP_DrStSWDTC_raw32_minval
      link override Signal_Override/_ovrdflg: Value=KOUTP_DrStSWDTC_raw32_ovrdflg
      link override Signal_Override/_ovrdval: Value=KOUTP_DrStSWDTC_raw32_ovrdval
  VDDM_EDriveSysErr_VCUErrTmp_flg_Inproc : FVT_lib/outp/OverrideAndLimit  SystemSampleTime=-1  VariantActivationTime=update diagram  Latency=0  AutoFrameSizeCalculation=off
      link override Signal_Limit/_maxval: Value=KOUTP_EDriveSysErr_VCUErrTmp_flg_maxval
      link override Signal_Limit/_minval: Value=KOUTP_EDriveSysErr_VCUErrTmp_flg_minval
      link override Signal_Override/_ovrdflg: Value=KOUTP_EDriveSysErr_VCUErrTmp_flg_ovrdflg
      link override Signal_Override/_ovrdval: Value=KOUTP_EDriveSysErr_VCUErrTmp_flg_ovrdval
  VDDM_EPBLockTODTC_raw32_Inproc : FVT_lib/outp/OverrideAndLimit  SystemSampleTime=-1  VariantActivationTime=update diagram  Latency=0  AutoFrameSizeCalculation=off
      link override Signal_Limit/_maxval: Value=KOUTP_EPBLockTODTC_raw32_maxval
      link override Signal_Limit/_minval: Value=KOUTP_EPBLockTODTC_raw32_minval
      link override Signal_Override/_ovrdflg: Value=KOUTP_EPBLockTODTC_raw32_ovrdflg
      link override Signal_Override/_ovrdval: Value=KOUTP_EPBLockTODTC_raw32_ovrdval
  VDDM_EPBUnlockTODTC_raw32_Inproc : FVT_lib/outp/OverrideAndLimit  SystemSampleTime=-1  VariantActivationTime=update diagram  Latency=0  AutoFrameSizeCalculation=off
      link override Signal_Limit/_maxval: Value=KOUTP_EPBUnlockTODTC_raw32_maxval
      link override Signal_Limit/_minval: Value=KOUTP_EPBUnlockTODTC_raw32_minval
      link override Signal_Override/_ovrdflg: Value=KOUTP_EPBUnlockTODTC_raw32_ovrdflg
      link override Signal_Override/_ovrdval: Value=KOUTP_EPBUnlockTODTC_raw32_ovrdval
  VDDM_ESC1CSErrDTC_raw32_Inproc : FVT_lib/outp/OverrideAndLimit  SystemSampleTime=-1  VariantActivationTime=update diagram  Latency=0  AutoFrameSizeCalculation=off
      link override Signal_Limit/_maxval: Value=KOUTP_ESC1CSErrDTC_raw32_maxval
      link override Signal_Limit/_minval: Value=KOUTP_ESC1CSErrDTC_raw32_minval
      link override Signal_Override/_ovrdflg: Value=KOUTP_ESC1CSErrDTC_raw32_ovrdflg
      link override Signal_Override/_ovrdval: Value=KOUTP_ESC1CSErrDTC_raw32_ovrdval
  VDDM_ESC1NoComDTC_raw32_Inproc : FVT_lib/outp/OverrideAndLimit  SystemSampleTime=-1  VariantActivationTime=update diagram  Latency=0  AutoFrameSizeCalculation=off
      link override Signal_Limit/_maxval: Value=KOUTP_ESC1NoComDTC_raw32_maxval
      link override Signal_Limit/_minval: Value=KOUTP_ESC1NoComDTC_raw32_minval
      link override Signal_Override/_ovrdflg: Value=KOUTP_ESC1NoComDTC_raw32_ovrdflg
      link override Signal_Override/_ovrdval: Value=KOUTP_ESC1NoComDTC_raw32_ovrdval
  VDDM_ESC1RCErrDTC_raw32_Inproc : FVT_lib/outp/OverrideAndLimit  SystemSampleTime=-1  VariantActivationTime=update diagram  Latency=0  AutoFrameSizeCalculation=off
      link override Signal_Limit/_maxval: Value=KOUTP_ESC1RCErrDTC_raw32_maxval
      link override Signal_Limit/_minval: Value=KOUTP_ESC1RCErrDTC_raw32_minval
      link override Signal_Override/_ovrdflg: Value=KOUTP_ESC1RCErrDTC_raw32_ovrdflg
      link override Signal_Override/_ovrdval: Value=KOUTP_ESC1RCErrDTC_raw32_ovrdval
  VDDM_ESC5CSErrDTC_raw32_Inproc : FVT_lib/outp/OverrideAndLimit  SystemSampleTime=-1  VariantActivationTime=update diagram  Latency=0  AutoFrameSizeCalculation=off
      link override Signal_Limit/_maxval: Value=KOUTP_ESC5CSErrDTC_raw32_maxval
      link override Signal_Limit/_minval: Value=KOUTP_ESC5CSErrDTC_raw32_minval
      link override Signal_Override/_ovrdflg: Value=KOUTP_ESC5CSErrDTC_raw32_ovrdflg
      link override Signal_Override/_ovrdval: Value=KOUTP_ESC5CSErrDTC_raw32_ovrdval
  VDDM_ESC5NoComDTC_raw32_Inproc : FVT_lib/outp/OverrideAndLimit  SystemSampleTime=-1  VariantActivationTime=update diagram  Latency=0  AutoFrameSizeCalculation=off
      link override Signal_Limit/_maxval: Value=KOUTP_ESC5NoComDTC_raw32_maxval
      link override Signal_Limit/_minval: Value=KOUTP_ESC5NoComDTC_raw32_minval
      link override Signal_Override/_ovrdflg: Value=KOUTP_ESC5NoComDTC_raw32_ovrdflg
      link override Signal_Override/_ovrdval: Value=KOUTP_ESC5NoComDTC_raw32_ovrdval
  VDDM_ESC5RCErrDTC_raw32_Inproc : FVT_lib/outp/OverrideAndLimit  SystemSampleTime=-1  VariantActivationTime=update diagram  Latency=0  AutoFrameSizeCalculation=off
      link override Signal_Limit/_maxval: Value=KOUTP_ESC5RCErrDTC_raw32_maxval
      link override Signal_Limit/_minval: Value=KOUTP_ESC5RCErrDTC_raw32_minval
      link override Signal_Override/_ovrdflg: Value=KOUTP_ESC5RCErrDTC_raw32_ovrdflg
      link override Signal_Override/_ovrdval: Value=KOUTP_ESC5RCErrDTC_raw32_ovrdval
  VDDM_ESC7CSErrDTC_raw32_Inproc : FVT_lib/outp/OverrideAndLimit  SystemSampleTime=-1  VariantActivationTime=update diagram  Latency=0  AutoFrameSizeCalculation=off
      link override Signal_Limit/_maxval: Value=KOUTP_ESC7CSErrDTC_raw32_maxval
      link override Signal_Limit/_minval: Value=KOUTP_ESC7CSErrDTC_raw32_minval
      link override Signal_Override/_ovrdflg: Value=KOUTP_ESC7CSErrDTC_raw32_ovrdflg
      link override Signal_Override/_ovrdval: Value=KOUTP_ESC7CSErrDTC_raw32_ovrdval
  VDDM_ESC7NoComDTC_raw32_Inproc : FVT_lib/outp/OverrideAndLimit  SystemSampleTime=-1  VariantActivationTime=update diagram  Latency=0  AutoFrameSizeCalculation=off
      link override Signal_Limit/_maxval: Value=KOUTP_ESC7NoComDTC_raw32_maxval
      link override Signal_Limit/_minval: Value=KOUTP_ESC7NoComDTC_raw32_minval
      link override Signal_Override/_ovrdflg: Value=KOUTP_ESC7NoComDTC_raw32_ovrdflg
      link override Signal_Override/_ovrdval: Value=KOUTP_ESC7NoComDTC_raw32_ovrdval
  VDDM_ESC7RCErrDTC_raw32_Inproc : FVT_lib/outp/OverrideAndLimit  SystemSampleTime=-1  VariantActivationTime=update diagram  Latency=0  AutoFrameSizeCalculation=off
      link override Signal_Limit/_maxval: Value=KOUTP_ESC7RCErrDTC_raw32_maxval
      link override Signal_Limit/_minval: Value=KOUTP_ESC7RCErrDTC_raw32_minval
      link override Signal_Override/_ovrdflg: Value=KOUTP_ESC7RCErrDTC_raw32_ovrdflg
      link override Signal_Override/_ovrdval: Value=KOUTP_ESC7RCErrDTC_raw32_ovrdval
  VDDM_EnterNewOperCyc_flg_Inproc : FVT_lib/outp/OverrideAndLimit  SystemSampleTime=-1  VariantActivationTime=update diagram  Latency=0  AutoFrameSizeCalculation=off
      link override Signal_Limit/_maxval: Value=KOUTP_EnterNewOperCyc_flg_maxval
      link override Signal_Limit/_minval: Value=KOUTP_EnterNewOperCyc_flg_minval
      link override Signal_Override/_ovrdflg: Value=KOUTP_EnterNewOperCyc_flg_ovrdflg
      link override Signal_Override/_ovrdval: Value=KOUTP_EnterNewOperCyc_flg_ovrdval
  VDDM_FCLUSSDTC_raw32_Inproc : FVT_lib/outp/OverrideAndLimit  SystemSampleTime=-1  VariantActivationTime=update diagram  Latency=0  AutoFrameSizeCalculation=off
      link override Signal_Limit/_maxval: Value=KOUTP_FCLUSSDTC_raw32_maxval
      link override Signal_Limit/_minval: Value=KOUTP_FCLUSSDTC_raw32_minval
      link override Signal_Override/_ovrdflg: Value=KOUTP_FCLUSSDTC_raw32_ovrdflg
      link override Signal_Override/_ovrdval: Value=KOUTP_FCLUSSDTC_raw32_ovrdval
  VDDM_FCM2CSErrDTC_raw32_Inproc : FVT_lib/outp/OverrideAndLimit  SystemSampleTime=-1  VariantActivationTime=update diagram  Latency=0  AutoFrameSizeCalculation=off
      link override Signal_Limit/_maxval: Value=KOUTP_FCM2CSErrDTC_raw32_maxval
      link override Signal_Limit/_minval: Value=KOUTP_FCM2CSErrDTC_raw32_minval
      link override Signal_Override/_ovrdflg: Value=KOUTP_FCM2CSErrDTC_raw32_ovrdflg
      link override Signal_Override/_ovrdval: Value=KOUTP_FCM2CSErrDTC_raw32_ovrdval
  VDDM_FCM2NoComDTC_raw32_Inproc : FVT_lib/outp/OverrideAndLimit  SystemSampleTime=-1  VariantActivationTime=update diagram  Latency=0  AutoFrameSizeCalculation=off
      link override Signal_Limit/_maxval: Value=KOUTP_FCM2NoComDTC_raw32_maxval
      link override Signal_Limit/_minval: Value=KOUTP_FCM2NoComDTC_raw32_minval
      link override Signal_Override/_ovrdflg: Value=KOUTP_FCM2NoComDTC_raw32_ovrdflg
      link override Signal_Override/_ovrdval: Value=KOUTP_FCM2NoComDTC_raw32_ovrdval
  VDDM_FCM2RCErrDTC_raw32_Inproc : FVT_lib/outp/OverrideAndLimit  SystemSampleTime=-1  VariantActivationTime=update diagram  Latency=0  AutoFrameSizeCalculation=off
      link override Signal_Limit/_maxval: Value=KOUTP_FCM2RCErrDTC_raw32_maxval
      link override Signal_Limit/_minval: Value=KOUTP_FCM2RCErrDTC_raw32_minval
      link override Signal_Override/_ovrdflg: Value=KOUTP_FCM2RCErrDTC_raw32_ovrdflg
      link override Signal_Override/_ovrdval: Value=KOUTP_FCM2RCErrDTC_raw32_ovrdval
  VDDM_FCM3CSErrDTC_raw32_Inproc : FVT_lib/outp/OverrideAndLimit  SystemSampleTime=-1  VariantActivationTime=update diagram  Latency=0  AutoFrameSizeCalculation=off
      link override Signal_Limit/_maxval: Value=KOUTP_FCM3CSErrDTC_raw32_maxval
      link override Signal_Limit/_minval: Value=KOUTP_FCM3CSErrDTC_raw32_minval
      link override Signal_Override/_ovrdflg: Value=KOUTP_FCM3CSErrDTC_raw32_ovrdflg
      link override Signal_Override/_ovrdval: Value=KOUTP_FCM3CSErrDTC_raw32_ovrdval
  VDDM_FCM3NoComDTC_raw32_Inproc : FVT_lib/outp/OverrideAndLimit  SystemSampleTime=-1  VariantActivationTime=update diagram  Latency=0  AutoFrameSizeCalculation=off
      link override Signal_Limit/_maxval: Value=KOUTP_FCM3NoComDTC_raw32_maxval
      link override Signal_Limit/_minval: Value=KOUTP_FCM3NoComDTC_raw32_minval
      link override Signal_Override/_ovrdflg: Value=KOUTP_FCM3NoComDTC_raw32_ovrdflg
      link override Signal_Override/_ovrdval: Value=KOUTP_FCM3NoComDTC_raw32_ovrdval
  VDDM_FCM3RCErrDTC_raw32_Inproc : FVT_lib/outp/OverrideAndLimit  SystemSampleTime=-1  VariantActivationTime=update diagram  Latency=0  AutoFrameSizeCalculation=off
      link override Signal_Limit/_maxval: Value=KOUTP_FCM3RCErrDTC_raw32_maxval
      link override Signal_Limit/_minval: Value=KOUTP_FCM3RCErrDTC_raw32_minval
      link override Signal_Override/_ovrdflg: Value=KOUTP_FCM3RCErrDTC_raw32_ovrdflg
      link override Signal_Override/_ovrdval: Value=KOUTP_FCM3RCErrDTC_raw32_ovrdval
  VDDM_FCM4CSErrDTC_raw32_Inproc : FVT_lib/outp/OverrideAndLimit  SystemSampleTime=-1  VariantActivationTime=update diagram  Latency=0  AutoFrameSizeCalculation=off
      link override Signal_Limit/_maxval: Value=KOUTP_FCM4CSErrDTC_raw32_maxval
      link override Signal_Limit/_minval: Value=KOUTP_FCM4CSErrDTC_raw32_minval
      link override Signal_Override/_ovrdflg: Value=KOUTP_FCM4CSErrDTC_raw32_ovrdflg
      link override Signal_Override/_ovrdval: Value=KOUTP_FCM4CSErrDTC_raw32_ovrdval
  VDDM_FCM4NoComDTC_raw32_Inproc : FVT_lib/outp/OverrideAndLimit  SystemSampleTime=-1  VariantActivationTime=update diagram  Latency=0  AutoFrameSizeCalculation=off
      link override Signal_Limit/_maxval: Value=KOUTP_FCM4NoComDTC_raw32_maxval
      link override Signal_Limit/_minval: Value=KOUTP_FCM4NoComDTC_raw32_minval
      link override Signal_Override/_ovrdflg: Value=KOUTP_FCM4NoComDTC_raw32_ovrdflg
      link override Signal_Override/_ovrdval: Value=KOUTP_FCM4NoComDTC_raw32_ovrdval
  VDDM_FCM5CSErrDTC_raw32_Inproc : FVT_lib/outp/OverrideAndLimit  SystemSampleTime=-1  VariantActivationTime=update diagram  Latency=0  AutoFrameSizeCalculation=off
      link override Signal_Limit/_maxval: Value=KOUTP_FCM5CSErrDTC_raw32_maxval
      link override Signal_Limit/_minval: Value=KOUTP_FCM5CSErrDTC_raw32_minval
      link override Signal_Override/_ovrdflg: Value=KOUTP_FCM5CSErrDTC_raw32_ovrdflg
      link override Signal_Override/_ovrdval: Value=KOUTP_FCM5CSErrDTC_raw32_ovrdval
  VDDM_FCM5NoComDTC_raw32_Inproc : FVT_lib/outp/OverrideAndLimit  SystemSampleTime=-1  VariantActivationTime=update diagram  Latency=0  AutoFrameSizeCalculation=off
      link override Signal_Limit/_maxval: Value=KOUTP_FCM5NoComDTC_raw32_maxval
      link override Signal_Limit/_minval: Value=KOUTP_FCM5NoComDTC_raw32_minval
      link override Signal_Override/_ovrdflg: Value=KOUTP_FCM5NoComDTC_raw32_ovrdflg
      link override Signal_Override/_ovrdval: Value=KOUTP_FCM5NoComDTC_raw32_ovrdval
  VDDM_FCMACCSigErrDetDTC_raw32_Inproc : FVT_lib/outp/OverrideAndLimit  SystemSampleTime=-1  VariantActivationTime=update diagram  Latency=0  AutoFrameSizeCalculation=off
      link override Signal_Limit/_maxval: Value=KOUTP_FCMACCSigErrDetDTC_raw32_maxval
      link override Signal_Limit/_minval: Value=KOUTP_FCMACCSigErrDetDTC_raw32_minval
      link override Signal_Override/_ovrdflg: Value=KOUTP_FCMACCSigErrDetDTC_raw32_ovrdflg
      link override Signal_Override/_ovrdval: Value=KOUTP_FCMACCSigErrDetDTC_raw32_ovrdval
  VDDM_FCRUSSDTC_raw32_Inproc : FVT_lib/outp/OverrideAndLimit  SystemSampleTime=-1  VariantActivationTime=update diagram  Latency=0  AutoFrameSizeCalculation=off
      link override Signal_Limit/_maxval: Value=KOUTP_FCRUSSDTC_raw32_maxval
      link override Signal_Limit/_minval: Value=KOUTP_FCRUSSDTC_raw32_minval
      link override Signal_Override/_ovrdflg: Value=KOUTP_FCRUSSDTC_raw32_ovrdflg
      link override Signal_Override/_ovrdval: Value=KOUTP_FCRUSSDTC_raw32_ovrdval
  VDDM_FLDoorSWDTC_raw32_Inproc : FVT_lib/outp/OverrideAndLimit  SystemSampleTime=-1  VariantActivationTime=update diagram  Latency=0  AutoFrameSizeCalculation=off
      link override Signal_Limit/_maxval: Value=KOUTP_FLDoorSWDTC_raw32_maxval
      link override Signal_Limit/_minval: Value=KOUTP_FLDoorSWDTC_raw32_minval
      link override Signal_Override/_ovrdflg: Value=KOUTP_FLDoorSWDTC_raw32_ovrdflg
      link override Signal_Override/_ovrdval: Value=KOUTP_FLDoorSWDTC_raw32_ovrdval
  VDDM_FLLUSSDTC_raw32_Inproc : FVT_lib/outp/OverrideAndLimit  SystemSampleTime=-1  VariantActivationTime=update diagram  Latency=0  AutoFrameSizeCalculation=off
      link override Signal_Limit/_maxval: Value=KOUTP_FLLUSSDTC_raw32_maxval
      link override Signal_Limit/_minval: Value=KOUTP_FLLUSSDTC_raw32_minval
      link override Signal_Override/_ovrdflg: Value=KOUTP_FLLUSSDTC_raw32_ovrdflg
      link override Signal_Override/_ovrdval: Value=KOUTP_FLLUSSDTC_raw32_ovrdval
  VDDM_FLRUSSDTC_raw32_Inproc : FVT_lib/outp/OverrideAndLimit  SystemSampleTime=-1  VariantActivationTime=update diagram  Latency=0  AutoFrameSizeCalculation=off
      link override Signal_Limit/_maxval: Value=KOUTP_FLRUSSDTC_raw32_maxval
      link override Signal_Limit/_minval: Value=KOUTP_FLRUSSDTC_raw32_minval
      link override Signal_Override/_ovrdflg: Value=KOUTP_FLRUSSDTC_raw32_ovrdflg
      link override Signal_Override/_ovrdval: Value=KOUTP_FLRUSSDTC_raw32_ovrdval
  VDDM_FMLUSSDTC_raw32_Inproc : FVT_lib/outp/OverrideAndLimit  SystemSampleTime=-1  VariantActivationTime=update diagram  Latency=0  AutoFrameSizeCalculation=off
      link override Signal_Limit/_maxval: Value=KOUTP_FMLUSSDTC_raw32_maxval
      link override Signal_Limit/_minval: Value=KOUTP_FMLUSSDTC_raw32_minval
      link override Signal_Override/_ovrdflg: Value=KOUTP_FMLUSSDTC_raw32_ovrdflg
      link override Signal_Override/_ovrdval: Value=KOUTP_FMLUSSDTC_raw32_ovrdval
  VDDM_FMRUSSDTC_raw32_Inproc : FVT_lib/outp/OverrideAndLimit  SystemSampleTime=-1  VariantActivationTime=update diagram  Latency=0  AutoFrameSizeCalculation=off
      link override Signal_Limit/_maxval: Value=KOUTP_FMRUSSDTC_raw32_maxval
      link override Signal_Limit/_minval: Value=KOUTP_FMRUSSDTC_raw32_minval
      link override Signal_Override/_ovrdflg: Value=KOUTP_FMRUSSDTC_raw32_ovrdflg
      link override Signal_Override/_ovrdval: Value=KOUTP_FMRUSSDTC_raw32_ovrdval
  VDDM_FRDoorSWDTC_raw32_Inproc : FVT_lib/outp/OverrideAndLimit  SystemSampleTime=-1  VariantActivationTime=update diagram  Latency=0  AutoFrameSizeCalculation=off
      link override Signal_Limit/_maxval: Value=KOUTP_FRDoorSWDTC_raw32_maxval
      link override Signal_Limit/_minval: Value=KOUTP_FRDoorSWDTC_raw32_minval
      link override Signal_Override/_ovrdflg: Value=KOUTP_FRDoorSWDTC_raw32_ovrdflg
      link override Signal_Override/_ovrdval: Value=KOUTP_FRDoorSWDTC_raw32_ovrdval
  VDDM_FrMCUSigErrDetDTC_raw32_Inproc : FVT_lib/outp/OverrideAndLimit  SystemSampleTime=-1  VariantActivationTime=update diagram  Latency=0  AutoFrameSizeCalculation=off
      link override Signal_Limit/_maxval: Value=KOUTP_FrMCUSigErrDetDTC_raw32_maxval
      link override Signal_Limit/_minval: Value=KOUTP_FrMCUSigErrDetDTC_raw32_minval
      link override Signal_Override/_ovrdflg: Value=KOUTP_FrMCUSigErrDetDTC_raw32_ovrdflg
      link override Signal_Override/_ovrdval: Value=KOUTP_FrMCUSigErrDetDTC_raw32_ovrdval
  VDDM_FrMCUTqErrDTC_raw32_Inproc : FVT_lib/outp/OverrideAndLimit  SystemSampleTime=-1  VariantActivationTime=update diagram  Latency=0  AutoFrameSizeCalculation=off
      link override Signal_Limit/_maxval: Value=KOUTP_FrMCUTqErrDTC_raw32_maxval
      link override Signal_Limit/_minval: Value=KOUTP_FrMCUTqErrDTC_raw32_minval
      link override Signal_Override/_ovrdflg: Value=KOUTP_FrMCUTqErrDTC_raw32_ovrdflg
      link override Signal_Override/_ovrdval: Value=KOUTP_FrMCUTqErrDTC_raw32_ovrdval
  VDDM_HVB4PreDTC_raw32_Inproc : FVT_lib/outp/OverrideAndLimit  SystemSampleTime=-1  VariantActivationTime=update diagram  Latency=0  AutoFrameSizeCalculation=off
      link override Signal_Limit/_maxval: Value=KOUTP_HVB4PreDTC_raw32_maxval
      link override Signal_Limit/_minval: Value=KOUTP_HVB4PreDTC_raw32_minval
      link override Signal_Override/_ovrdflg: Value=KOUTP_HVB4PreDTC_raw32_ovrdflg
      link override Signal_Override/_ovrdval: Value=KOUTP_HVB4PreDTC_raw32_ovrdval
  VDDM_HVRlyCloDTC_raw32_Inproc : FVT_lib/outp/OverrideAndLimit  SystemSampleTime=-1  VariantActivationTime=update diagram  Latency=0  AutoFrameSizeCalculation=off
      link override Signal_Limit/_maxval: Value=KOUTP_HVRlyCloDTC_raw32_maxval
      link override Signal_Limit/_minval: Value=KOUTP_HVRlyCloDTC_raw32_minval
      link override Signal_Override/_ovrdflg: Value=KOUTP_HVRlyCloDTC_raw32_ovrdflg
      link override Signal_Override/_ovrdval: Value=KOUTP_HVRlyCloDTC_raw32_ovrdval
  VDDM_HVRlyOpDTC_raw32_Inproc : FVT_lib/outp/OverrideAndLimit  SystemSampleTime=-1  VariantActivationTime=update diagram  Latency=0  AutoFrameSizeCalculation=off
      link override Signal_Limit/_maxval: Value=KOUTP_HVRlyOpDTC_raw32_maxval
      link override Signal_Limit/_minval: Value=KOUTP_HVRlyOpDTC_raw32_minval
      link override Signal_Override/_ovrdflg: Value=KOUTP_HVRlyOpDTC_raw32_ovrdflg
      link override Signal_Override/_ovrdval: Value=KOUTP_HVRlyOpDTC_raw32_ovrdval
  VDDM_HiLvSaChkDTC_raw32_Inproc : FVT_lib/outp/OverrideAndLimit  SystemSampleTime=-1  VariantActivationTime=update diagram  Latency=0  AutoFrameSizeCalculation=off
      link override Signal_Limit/_maxval: Value=KOUTP_HiLvSaChkDTC_raw32_maxval
      link override Signal_Limit/_minval: Value=KOUTP_HiLvSaChkDTC_raw32_minval
      link override Signal_Override/_ovrdflg: Value=KOUTP_HiLvSaChkDTC_raw32_ovrdflg
      link override Signal_Override/_ovrdval: Value=KOUTP_HiLvSaChkDTC_raw32_ovrdval
  VDDM_HoodSWDTC_raw32_Inproc : FVT_lib/outp/OverrideAndLimit  SystemSampleTime=-1  VariantActivationTime=update diagram  Latency=0  AutoFrameSizeCalculation=off
      link override Signal_Limit/_maxval: Value=KOUTP_HoodSWDTC_raw32_maxval
      link override Signal_Limit/_minval: Value=KOUTP_HoodSWDTC_raw32_minval
      link override Signal_Override/_ovrdflg: Value=KOUTP_HoodSWDTC_raw32_ovrdflg
      link override Signal_Override/_ovrdval: Value=KOUTP_HoodSWDTC_raw32_ovrdval
  VDDM_ISAMalfuncDetDTC_raw32_Inproc : FVT_lib/outp/OverrideAndLimit  SystemSampleTime=-1  VariantActivationTime=update diagram  Latency=0  AutoFrameSizeCalculation=off
      link override Signal_Limit/_maxval: Value=KOUTP_ISAMalfuncDetDTC_raw32_maxval
      link override Signal_Limit/_minval: Value=KOUTP_ISAMalfuncDetDTC_raw32_minval
      link override Signal_Override/_ovrdflg: Value=KOUTP_ISAMalfuncDetDTC_raw32_ovrdflg
      link override Signal_Override/_ovrdval: Value=KOUTP_ISAMalfuncDetDTC_raw32_ovrdval
  VDDM_IniLVLoDTC_raw32_Inproc : FVT_lib/outp/OverrideAndLimit  SystemSampleTime=-1  VariantActivationTime=update diagram  Latency=0  AutoFrameSizeCalculation=off
      link override Signal_Limit/_maxval: Value=KOUTP_IniLVLoDTC_raw32_maxval
      link override Signal_Limit/_minval: Value=KOUTP_IniLVLoDTC_raw32_minval
      link override Signal_Override/_ovrdflg: Value=KOUTP_IniLVLoDTC_raw32_ovrdflg
      link override Signal_Override/_ovrdval: Value=KOUTP_IniLVLoDTC_raw32_ovrdval
  VDDM_KeyAuthDTC_raw32_Inproc : FVT_lib/outp/OverrideAndLimit  SystemSampleTime=-1  VariantActivationTime=update diagram  Latency=0  AutoFrameSizeCalculation=off
      link override Signal_Limit/_maxval: Value=KOUTP_KeyAuthDTC_raw32_maxval
      link override Signal_Limit/_minval: Value=KOUTP_KeyAuthDTC_raw32_minval
      link override Signal_Override/_ovrdflg: Value=KOUTP_KeyAuthDTC_raw32_ovrdflg
      link override Signal_Override/_ovrdval: Value=KOUTP_KeyAuthDTC_raw32_ovrdval
  VDDM_LFBatwarnDTC_raw32_Inproc : FVT_lib/outp/OverrideAndLimit  SystemSampleTime=-1  VariantActivationTime=update diagram  Latency=0  AutoFrameSizeCalculation=off
      link override Signal_Limit/_maxval: Value=KOUTP_LFBatwarnDTC_raw32_maxval
      link override Signal_Limit/_minval: Value=KOUTP_LFBatwarnDTC_raw32_minval
      link override Signal_Override/_ovrdflg: Value=KOUTP_LFBatwarnDTC_raw32_ovrdflg
      link override Signal_Override/_ovrdval: Value=KOUTP_LFBatwarnDTC_raw32_ovrdval
  VDDM_LFPressIndiDTC_raw32_Inproc : FVT_lib/outp/OverrideAndLimit  SystemSampleTime=-1  VariantActivationTime=update diagram  Latency=0  AutoFrameSizeCalculation=off
      link override Signal_Limit/_maxval: Value=KOUTP_LFPressIndiDTC_raw32_maxval
      link override Signal_Limit/_minval: Value=KOUTP_LFPressIndiDTC_raw32_minval
      link override Signal_Override/_ovrdflg: Value=KOUTP_LFPressIndiDTC_raw32_ovrdflg
      link override Signal_Override/_ovrdval: Value=KOUTP_LFPressIndiDTC_raw32_ovrdval
  VDDM_LFSensorFailDTC_raw32_Inproc : FVT_lib/outp/OverrideAndLimit  SystemSampleTime=-1  VariantActivationTime=update diagram  Latency=0  AutoFrameSizeCalculation=off
      link override Signal_Limit/_maxval: Value=KOUTP_LFSensorFailDTC_raw32_maxval
      link override Signal_Limit/_minval: Value=KOUTP_LFSensorFailDTC_raw32_minval
      link override Signal_Override/_ovrdflg: Value=KOUTP_LFSensorFailDTC_raw32_ovrdflg
      link override Signal_Override/_ovrdval: Value=KOUTP_LFSensorFailDTC_raw32_ovrdval
  VDDM_LFWheelTmpHighDTC_raw32_Inproc : FVT_lib/outp/OverrideAndLimit  SystemSampleTime=-1  VariantActivationTime=update diagram  Latency=0  AutoFrameSizeCalculation=off
      link override Signal_Limit/_maxval: Value=KOUTP_LFWheelTmpHighDTC_raw32_maxval
      link override Signal_Limit/_minval: Value=KOUTP_LFWheelTmpHighDTC_raw32_minval
      link override Signal_Override/_ovrdflg: Value=KOUTP_LFWheelTmpHighDTC_raw32_ovrdflg
      link override Signal_Override/_ovrdval: Value=KOUTP_LFWheelTmpHighDTC_raw32_ovrdval
  VDDM_LRBatwarnDTC_raw32_Inproc : FVT_lib/outp/OverrideAndLimit  SystemSampleTime=-1  VariantActivationTime=update diagram  Latency=0  AutoFrameSizeCalculation=off
      link override Signal_Limit/_maxval: Value=KOUTP_LRBatwarnDTC_raw32_maxval
      link override Signal_Limit/_minval: Value=KOUTP_LRBatwarnDTC_raw32_minval
      link override Signal_Override/_ovrdflg: Value=KOUTP_LRBatwarnDTC_raw32_ovrdflg
      link override Signal_Override/_ovrdval: Value=KOUTP_LRBatwarnDTC_raw32_ovrdval
  VDDM_LRPressIndiDTC_raw32_Inproc : FVT_lib/outp/OverrideAndLimit  SystemSampleTime=-1  VariantActivationTime=update diagram  Latency=0  AutoFrameSizeCalculation=off
      link override Signal_Limit/_maxval: Value=KOUTP_LRPressIndiDTC_raw32_maxval
      link override Signal_Limit/_minval: Value=KOUTP_LRPressIndiDTC_raw32_minval
      link override Signal_Override/_ovrdflg: Value=KOUTP_LRPressIndiDTC_raw32_ovrdflg
      link override Signal_Override/_ovrdval: Value=KOUTP_LRPressIndiDTC_raw32_ovrdval
  VDDM_LRSensorFailDTC_raw32_Inproc : FVT_lib/outp/OverrideAndLimit  SystemSampleTime=-1  VariantActivationTime=update diagram  Latency=0  AutoFrameSizeCalculation=off
      link override Signal_Limit/_maxval: Value=KOUTP_LRSensorFailDTC_raw32_maxval
      link override Signal_Limit/_minval: Value=KOUTP_LRSensorFailDTC_raw32_minval
      link override Signal_Override/_ovrdflg: Value=KOUTP_LRSensorFailDTC_raw32_ovrdflg
      link override Signal_Override/_ovrdval: Value=KOUTP_LRSensorFailDTC_raw32_ovrdval
  VDDM_LRWheelTmpHighDTC_raw32_Inproc : FVT_lib/outp/OverrideAndLimit  SystemSampleTime=-1  VariantActivationTime=update diagram  Latency=0  AutoFrameSizeCalculation=off
      link override Signal_Limit/_maxval: Value=KOUTP_LRWheelTmpHighDTC_raw32_maxval
      link override Signal_Limit/_minval: Value=KOUTP_LRWheelTmpHighDTC_raw32_minval
      link override Signal_Override/_ovrdflg: Value=KOUTP_LRWheelTmpHighDTC_raw32_ovrdflg
      link override Signal_Override/_ovrdval: Value=KOUTP_LRWheelTmpHighDTC_raw32_ovrdval
  VDDM_LVSupHiDTC_raw32_Inproc : FVT_lib/outp/OverrideAndLimit  SystemSampleTime=-1  VariantActivationTime=update diagram  Latency=0  AutoFrameSizeCalculation=off
      link override Signal_Limit/_maxval: Value=KOUTP_LVSupHiDTC_raw32_maxval
      link override Signal_Limit/_minval: Value=KOUTP_LVSupHiDTC_raw32_minval
      link override Signal_Override/_ovrdflg: Value=KOUTP_LVSupHiDTC_raw32_ovrdflg
      link override Signal_Override/_ovrdval: Value=KOUTP_LVSupHiDTC_raw32_ovrdval
  VDDM_LVSupLoDTC_raw32_Inproc : FVT_lib/outp/OverrideAndLimit  SystemSampleTime=-1  VariantActivationTime=update diagram  Latency=0  AutoFrameSizeCalculation=off
      link override Signal_Limit/_maxval: Value=KOUTP_LVSupLoDTC_raw32_maxval
      link override Signal_Limit/_minval: Value=KOUTP_LVSupLoDTC_raw32_minval
      link override Signal_Override/_ovrdflg: Value=KOUTP_LVSupLoDTC_raw32_ovrdflg
      link override Signal_Override/_ovrdval: Value=KOUTP_LVSupLoDTC_raw32_ovrdval
  VDDM_LimpHomeActTmp_flg_Inproc : FVT_lib/outp/OverrideAndLimit  SystemSampleTime=-1  VariantActivationTime=update diagram  Latency=0  AutoFrameSizeCalculation=off
      link override Signal_Limit/_maxval: Value=KOUTP_LimpHomeActTmp_flg_maxval
      link override Signal_Limit/_minval: Value=KOUTP_LimpHomeActTmp_flg_minval
      link override Signal_Override/_ovrdflg: Value=KOUTP_LimpHomeActTmp_flg_ovrdflg
      link override Signal_Override/_ovrdval: Value=KOUTP_LimpHomeActTmp_flg_ovrdval
  VDDM_Lv1ErrDTC_raw32_Inproc : FVT_lib/outp/OverrideAndLimit  SystemSampleTime=-1  VariantActivationTime=update diagram  Latency=0  AutoFrameSizeCalculation=off
      link override Signal_Limit/_maxval: Value=KOUTP_Lv1ErrDTC_raw32_maxval
      link override Signal_Limit/_minval: Value=KOUTP_Lv1ErrDTC_raw32_minval
      link override Signal_Override/_ovrdflg: Value=KOUTP_Lv1ErrDTC_raw32_ovrdflg
      link override Signal_Override/_ovrdval: Value=KOUTP_Lv1ErrDTC_raw32_ovrdval
  VDDM_Lv2ErrDTC_raw32_Inproc : FVT_lib/outp/OverrideAndLimit  SystemSampleTime=-1  VariantActivationTime=update diagram  Latency=0  AutoFrameSizeCalculation=off
      link override Signal_Limit/_maxval: Value=KOUTP_Lv2ErrDTC_raw32_maxval
      link override Signal_Limit/_minval: Value=KOUTP_Lv2ErrDTC_raw32_minval
      link override Signal_Override/_ovrdflg: Value=KOUTP_Lv2ErrDTC_raw32_ovrdflg
      link override Signal_Override/_ovrdval: Value=KOUTP_Lv2ErrDTC_raw32_ovrdval
  VDDM_Lv3ErrDTC_raw32_Inproc : FVT_lib/outp/OverrideAndLimit  SystemSampleTime=-1  VariantActivationTime=update diagram  Latency=0  AutoFrameSizeCalculation=off
      link override Signal_Limit/_maxval: Value=KOUTP_Lv3ErrDTC_raw32_maxval
      link override Signal_Limit/_minval: Value=KOUTP_Lv3ErrDTC_raw32_minval
      link override Signal_Override/_ovrdflg: Value=KOUTP_Lv3ErrDTC_raw32_ovrdflg
      link override Signal_Override/_ovrdval: Value=KOUTP_Lv3ErrDTC_raw32_ovrdval
  VDDM_Lv4ErrDTC_raw32_Inproc : FVT_lib/outp/OverrideAndLimit  SystemSampleTime=-1  VariantActivationTime=update diagram  Latency=0  AutoFrameSizeCalculation=off
      link override Signal_Limit/_maxval: Value=KOUTP_Lv4ErrDTC_raw32_maxval
      link override Signal_Limit/_minval: Value=KOUTP_Lv4ErrDTC_raw32_minval
      link override Signal_Override/_ovrdflg: Value=KOUTP_Lv4ErrDTC_raw32_ovrdflg
      link override Signal_Override/_ovrdval: Value=KOUTP_Lv4ErrDTC_raw32_ovrdval
  VDDM_MCU4PreDTC_raw32_Inproc : FVT_lib/outp/OverrideAndLimit  SystemSampleTime=-1  VariantActivationTime=update diagram  Latency=0  AutoFrameSizeCalculation=off
      link override Signal_Limit/_maxval: Value=KOUTP_MCU4PreDTC_raw32_maxval
      link override Signal_Limit/_minval: Value=KOUTP_MCU4PreDTC_raw32_minval
      link override Signal_Override/_ovrdflg: Value=KOUTP_MCU4PreDTC_raw32_ovrdflg
      link override Signal_Override/_ovrdval: Value=KOUTP_MCU4PreDTC_raw32_ovrdval
  VDDM_MCUActDTC_raw32_Inproc : FVT_lib/outp/OverrideAndLimit  SystemSampleTime=-1  VariantActivationTime=update diagram  Latency=0  AutoFrameSizeCalculation=off
      link override Signal_Limit/_maxval: Value=KOUTP_MCUActDTC_raw32_maxval
      link override Signal_Limit/_minval: Value=KOUTP_MCUActDTC_raw32_minval
      link override Signal_Override/_ovrdflg: Value=KOUTP_MCUActDTC_raw32_ovrdflg
      link override Signal_Override/_ovrdval: Value=KOUTP_MCUActDTC_raw32_ovrdval
  VDDM_MCUDisDTC_raw32_Inproc : FVT_lib/outp/OverrideAndLimit  SystemSampleTime=-1  VariantActivationTime=update diagram  Latency=0  AutoFrameSizeCalculation=off
      link override Signal_Limit/_maxval: Value=KOUTP_MCUDisDTC_raw32_maxval
      link override Signal_Limit/_minval: Value=KOUTP_MCUDisDTC_raw32_minval
      link override Signal_Override/_ovrdflg: Value=KOUTP_MCUDisDTC_raw32_ovrdflg
      link override Signal_Override/_ovrdval: Value=KOUTP_MCUDisDTC_raw32_ovrdval
  VDDM_MCUF1CSErrDTC_raw32_Inproc : FVT_lib/outp/OverrideAndLimit  SystemSampleTime=-1  VariantActivationTime=update diagram  Latency=0  AutoFrameSizeCalculation=off
      link override Signal_Limit/_maxval: Value=KOUTP_MCUF1CSErrDTC_raw32_maxval
      link override Signal_Limit/_minval: Value=KOUTP_MCUF1CSErrDTC_raw32_minval
      link override Signal_Override/_ovrdflg: Value=KOUTP_MCUF1CSErrDTC_raw32_ovrdflg
      link override Signal_Override/_ovrdval: Value=KOUTP_MCUF1CSErrDTC_raw32_ovrdval
  VDDM_MCUF1NoComDTC_raw32_Inproc : FVT_lib/outp/OverrideAndLimit  SystemSampleTime=-1  VariantActivationTime=update diagram  Latency=0  AutoFrameSizeCalculation=off
      link override Signal_Limit/_maxval: Value=KOUTP_MCUF1NoComDTC_raw32_maxval
      link override Signal_Limit/_minval: Value=KOUTP_MCUF1NoComDTC_raw32_minval
      link override Signal_Override/_ovrdflg: Value=KOUTP_MCUF1NoComDTC_raw32_ovrdflg
      link override Signal_Override/_ovrdval: Value=KOUTP_MCUF1NoComDTC_raw32_ovrdval
  VDDM_MCUF1RCErrDTC_raw32_Inproc : FVT_lib/outp/OverrideAndLimit  SystemSampleTime=-1  VariantActivationTime=update diagram  Latency=0  AutoFrameSizeCalculation=off
      link override Signal_Limit/_maxval: Value=KOUTP_MCUF1RCErrDTC_raw32_maxval
      link override Signal_Limit/_minval: Value=KOUTP_MCUF1RCErrDTC_raw32_minval
      link override Signal_Override/_ovrdflg: Value=KOUTP_MCUF1RCErrDTC_raw32_ovrdflg
      link override Signal_Override/_ovrdval: Value=KOUTP_MCUF1RCErrDTC_raw32_ovrdval
  VDDM_MCUR1CSErrDTC_raw32_Inproc : FVT_lib/outp/OverrideAndLimit  SystemSampleTime=-1  VariantActivationTime=update diagram  Latency=0  AutoFrameSizeCalculation=off
      link override Signal_Limit/_maxval: Value=KOUTP_MCUR1CSErrDTC_raw32_maxval
      link override Signal_Limit/_minval: Value=KOUTP_MCUR1CSErrDTC_raw32_minval
      link override Signal_Override/_ovrdflg: Value=KOUTP_MCUR1CSErrDTC_raw32_ovrdflg
      link override Signal_Override/_ovrdval: Value=KOUTP_MCUR1CSErrDTC_raw32_ovrdval
  VDDM_MCUR1NoComDTC_raw32_Inproc : FVT_lib/outp/OverrideAndLimit  SystemSampleTime=-1  VariantActivationTime=update diagram  Latency=0  AutoFrameSizeCalculation=off
      link override Signal_Limit/_maxval: Value=KOUTP_MCUR1NoComDTC_raw32_maxval
      link override Signal_Limit/_minval: Value=KOUTP_MCUR1NoComDTC_raw32_minval
      link override Signal_Override/_ovrdflg: Value=KOUTP_MCUR1NoComDTC_raw32_ovrdflg
      link override Signal_Override/_ovrdval: Value=KOUTP_MCUR1NoComDTC_raw32_ovrdval
  VDDM_MCUR1RCErrDTC_raw32_Inproc : FVT_lib/outp/OverrideAndLimit  SystemSampleTime=-1  VariantActivationTime=update diagram  Latency=0  AutoFrameSizeCalculation=off
      link override Signal_Limit/_maxval: Value=KOUTP_MCUR1RCErrDTC_raw32_maxval
      link override Signal_Limit/_minval: Value=KOUTP_MCUR1RCErrDTC_raw32_minval
      link override Signal_Override/_ovrdflg: Value=KOUTP_MCUR1RCErrDTC_raw32_ovrdflg
      link override Signal_Override/_ovrdval: Value=KOUTP_MCUR1RCErrDTC_raw32_ovrdval
  VDDM_MSAMalfuncDetDTC_raw32_Inproc : FVT_lib/outp/OverrideAndLimit  SystemSampleTime=-1  VariantActivationTime=update diagram  Latency=0  AutoFrameSizeCalculation=off
      link override Signal_Limit/_maxval: Value=KOUTP_MSAMalfuncDetDTC_raw32_maxval
      link override Signal_Limit/_minval: Value=KOUTP_MSAMalfuncDetDTC_raw32_minval
      link override Signal_Override/_ovrdflg: Value=KOUTP_MSAMalfuncDetDTC_raw32_ovrdflg
      link override Signal_Override/_ovrdval: Value=KOUTP_MSAMalfuncDetDTC_raw32_ovrdval
  VDDM_MidLvSaChkDTC_raw32_Inproc : FVT_lib/outp/OverrideAndLimit  SystemSampleTime=-1  VariantActivationTime=update diagram  Latency=0  AutoFrameSizeCalculation=off
      link override Signal_Limit/_maxval: Value=KOUTP_MidLvSaChkDTC_raw32_maxval
      link override Signal_Limit/_minval: Value=KOUTP_MidLvSaChkDTC_raw32_minval
      link override Signal_Override/_ovrdflg: Value=KOUTP_MidLvSaChkDTC_raw32_ovrdflg
      link override Signal_Override/_ovrdval: Value=KOUTP_MidLvSaChkDTC_raw32_ovrdval
  VDDM_OBC4PreDTC_raw32_Inproc : FVT_lib/outp/OverrideAndLimit  SystemSampleTime=-1  VariantActivationTime=update diagram  Latency=0  AutoFrameSizeCalculation=off
      link override Signal_Limit/_maxval: Value=KOUTP_OBC4PreDTC_raw32_maxval
      link override Signal_Limit/_minval: Value=KOUTP_OBC4PreDTC_raw32_minval
      link override Signal_Override/_ovrdflg: Value=KOUTP_OBC4PreDTC_raw32_ovrdflg
      link override Signal_Override/_ovrdval: Value=KOUTP_OBC4PreDTC_raw32_ovrdval
  VDDM_ONtoRdyDTC_raw32_Inproc : FVT_lib/outp/OverrideAndLimit  SystemSampleTime=-1  VariantActivationTime=update diagram  Latency=0  AutoFrameSizeCalculation=off
      link override Signal_Limit/_maxval: Value=KOUTP_ONtoRdyDTC_raw32_maxval
      link override Signal_Limit/_minval: Value=KOUTP_ONtoRdyDTC_raw32_minval
      link override Signal_Override/_ovrdflg: Value=KOUTP_ONtoRdyDTC_raw32_ovrdflg
      link override Signal_Override/_ovrdval: Value=KOUTP_ONtoRdyDTC_raw32_ovrdval
  VDDM_RCLUSSDTC_raw32_Inproc : FVT_lib/outp/OverrideAndLimit  SystemSampleTime=-1  VariantActivationTime=update diagram  Latency=0  AutoFrameSizeCalculation=off
      link override Signal_Limit/_maxval: Value=KOUTP_RCLUSSDTC_raw32_maxval
      link override Signal_Limit/_minval: Value=KOUTP_RCLUSSDTC_raw32_minval
      link override Signal_Override/_ovrdflg: Value=KOUTP_RCLUSSDTC_raw32_ovrdflg
      link override Signal_Override/_ovrdval: Value=KOUTP_RCLUSSDTC_raw32_ovrdval
  VDDM_RCRUSSDTC_raw32_Inproc : FVT_lib/outp/OverrideAndLimit  SystemSampleTime=-1  VariantActivationTime=update diagram  Latency=0  AutoFrameSizeCalculation=off
      link override Signal_Limit/_maxval: Value=KOUTP_RCRUSSDTC_raw32_maxval
      link override Signal_Limit/_minval: Value=KOUTP_RCRUSSDTC_raw32_minval
      link override Signal_Override/_ovrdflg: Value=KOUTP_RCRUSSDTC_raw32_ovrdflg
      link override Signal_Override/_ovrdval: Value=KOUTP_RCRUSSDTC_raw32_ovrdval
  VDDM_RFBatwarnDTC_raw32_Inproc : FVT_lib/outp/OverrideAndLimit  SystemSampleTime=-1  VariantActivationTime=update diagram  Latency=0  AutoFrameSizeCalculation=off
      link override Signal_Limit/_maxval: Value=KOUTP_RFBatwarnDTC_raw32_maxval
      link override Signal_Limit/_minval: Value=KOUTP_RFBatwarnDTC_raw32_minval
      link override Signal_Override/_ovrdflg: Value=KOUTP_RFBatwarnDTC_raw32_ovrdflg
      link override Signal_Override/_ovrdval: Value=KOUTP_RFBatwarnDTC_raw32_ovrdval
  VDDM_RFPressIndiDTC_raw32_Inproc : FVT_lib/outp/OverrideAndLimit  SystemSampleTime=-1  VariantActivationTime=update diagram  Latency=0  AutoFrameSizeCalculation=off
      link override Signal_Limit/_maxval: Value=KOUTP_RFPressIndiDTC_raw32_maxval
      link override Signal_Limit/_minval: Value=KOUTP_RFPressIndiDTC_raw32_minval
      link override Signal_Override/_ovrdflg: Value=KOUTP_RFPressIndiDTC_raw32_ovrdflg
      link override Signal_Override/_ovrdval: Value=KOUTP_RFPressIndiDTC_raw32_ovrdval
  VDDM_RFSensorFailDTC_raw32_Inproc : FVT_lib/outp/OverrideAndLimit  SystemSampleTime=-1  VariantActivationTime=update diagram  Latency=0  AutoFrameSizeCalculation=off
      link override Signal_Limit/_maxval: Value=KOUTP_RFSensorFailDTC_raw32_maxval
      link override Signal_Limit/_minval: Value=KOUTP_RFSensorFailDTC_raw32_minval
      link override Signal_Override/_ovrdflg: Value=KOUTP_RFSensorFailDTC_raw32_ovrdflg
      link override Signal_Override/_ovrdval: Value=KOUTP_RFSensorFailDTC_raw32_ovrdval
  VDDM_RFWheelTmpHighDTC_raw32_Inproc : FVT_lib/outp/OverrideAndLimit  SystemSampleTime=-1  VariantActivationTime=update diagram  Latency=0  AutoFrameSizeCalculation=off
      link override Signal_Limit/_maxval: Value=KOUTP_RFWheelTmpHighDTC_raw32_maxval
      link override Signal_Limit/_minval: Value=KOUTP_RFWheelTmpHighDTC_raw32_minval
      link override Signal_Override/_ovrdflg: Value=KOUTP_RFWheelTmpHighDTC_raw32_ovrdflg
      link override Signal_Override/_ovrdval: Value=KOUTP_RFWheelTmpHighDTC_raw32_ovrdval
  VDDM_RLDoorSWDTC_raw32_Inproc : FVT_lib/outp/OverrideAndLimit  SystemSampleTime=-1  VariantActivationTime=update diagram  Latency=0  AutoFrameSizeCalculation=off
      link override Signal_Limit/_maxval: Value=KOUTP_RLDoorSWDTC_raw32_maxval
      link override Signal_Limit/_minval: Value=KOUTP_RLDoorSWDTC_raw32_minval
      link override Signal_Override/_ovrdflg: Value=KOUTP_RLDoorSWDTC_raw32_ovrdflg
      link override Signal_Override/_ovrdval: Value=KOUTP_RLDoorSWDTC_raw32_ovrdval
  VDDM_RLLUSSDTC_raw32_Inproc : FVT_lib/outp/OverrideAndLimit  SystemSampleTime=-1  VariantActivationTime=update diagram  Latency=0  AutoFrameSizeCalculation=off
      link override Signal_Limit/_maxval: Value=KOUTP_RLLUSSDTC_raw32_maxval
      link override Signal_Limit/_minval: Value=KOUTP_RLLUSSDTC_raw32_minval
      link override Signal_Override/_ovrdflg: Value=KOUTP_RLLUSSDTC_raw32_ovrdflg
      link override Signal_Override/_ovrdval: Value=KOUTP_RLLUSSDTC_raw32_ovrdval
  VDDM_RLRUSSDTC_raw32_Inproc : FVT_lib/outp/OverrideAndLimit  SystemSampleTime=-1  VariantActivationTime=update diagram  Latency=0  AutoFrameSizeCalculation=off
      link override Signal_Limit/_maxval: Value=KOUTP_RLRUSSDTC_raw32_maxval
      link override Signal_Limit/_minval: Value=KOUTP_RLRUSSDTC_raw32_minval
      link override Signal_Override/_ovrdflg: Value=KOUTP_RLRUSSDTC_raw32_ovrdflg
      link override Signal_Override/_ovrdval: Value=KOUTP_RLRUSSDTC_raw32_ovrdval
  VDDM_RMLUSSDTC_raw32_Inproc : FVT_lib/outp/OverrideAndLimit  SystemSampleTime=-1  VariantActivationTime=update diagram  Latency=0  AutoFrameSizeCalculation=off
      link override Signal_Limit/_maxval: Value=KOUTP_RMLUSSDTC_raw32_maxval
      link override Signal_Limit/_minval: Value=KOUTP_RMLUSSDTC_raw32_minval
      link override Signal_Override/_ovrdflg: Value=KOUTP_RMLUSSDTC_raw32_ovrdflg
      link override Signal_Override/_ovrdval: Value=KOUTP_RMLUSSDTC_raw32_ovrdval
  VDDM_RMRUSSDTC_raw32_Inproc : FVT_lib/outp/OverrideAndLimit  SystemSampleTime=-1  VariantActivationTime=update diagram  Latency=0  AutoFrameSizeCalculation=off
      link override Signal_Limit/_maxval: Value=KOUTP_RMRUSSDTC_raw32_maxval
      link override Signal_Limit/_minval: Value=KOUTP_RMRUSSDTC_raw32_minval
      link override Signal_Override/_ovrdflg: Value=KOUTP_RMRUSSDTC_raw32_ovrdflg
      link override Signal_Override/_ovrdval: Value=KOUTP_RMRUSSDTC_raw32_ovrdval
  VDDM_RRBatwarnDTC_raw32_Inproc : FVT_lib/outp/OverrideAndLimit  SystemSampleTime=-1  VariantActivationTime=update diagram  Latency=0  AutoFrameSizeCalculation=off
      link override Signal_Limit/_maxval: Value=KOUTP_RRBatwarnDTC_raw32_maxval
      link override Signal_Limit/_minval: Value=KOUTP_RRBatwarnDTC_raw32_minval
      link override Signal_Override/_ovrdflg: Value=KOUTP_RRBatwarnDTC_raw32_ovrdflg
      link override Signal_Override/_ovrdval: Value=KOUTP_RRBatwarnDTC_raw32_ovrdval
  VDDM_RRDoorSWDTC_raw32_Inproc : FVT_lib/outp/OverrideAndLimit  SystemSampleTime=-1  VariantActivationTime=update diagram  Latency=0  AutoFrameSizeCalculation=off
      link override Signal_Limit/_maxval: Value=KOUTP_RRDoorSWDTC_raw32_maxval
      link override Signal_Limit/_minval: Value=KOUTP_RRDoorSWDTC_raw32_minval
      link override Signal_Override/_ovrdflg: Value=KOUTP_RRDoorSWDTC_raw32_ovrdflg
      link override Signal_Override/_ovrdval: Value=KOUTP_RRDoorSWDTC_raw32_ovrdval
  VDDM_RRPressIndiDTC_raw32_Inproc : FVT_lib/outp/OverrideAndLimit  SystemSampleTime=-1  VariantActivationTime=update diagram  Latency=0  AutoFrameSizeCalculation=off
      link override Signal_Limit/_maxval: Value=KOUTP_RRPressIndiDTC_raw32_maxval
      link override Signal_Limit/_minval: Value=KOUTP_RRPressIndiDTC_raw32_minval
      link override Signal_Override/_ovrdflg: Value=KOUTP_RRPressIndiDTC_raw32_ovrdflg
      link override Signal_Override/_ovrdval: Value=KOUTP_RRPressIndiDTC_raw32_ovrdval
  VDDM_RRSensorFailDTC_raw32_Inproc : FVT_lib/outp/OverrideAndLimit  SystemSampleTime=-1  VariantActivationTime=update diagram  Latency=0  AutoFrameSizeCalculation=off
      link override Signal_Limit/_maxval: Value=KOUTP_RRSensorFailDTC_raw32_maxval
      link override Signal_Limit/_minval: Value=KOUTP_RRSensorFailDTC_raw32_minval
      link override Signal_Override/_ovrdflg: Value=KOUTP_RRSensorFailDTC_raw32_ovrdflg
      link override Signal_Override/_ovrdval: Value=KOUTP_RRSensorFailDTC_raw32_ovrdval
  VDDM_RRWheelTmpHighDTC_raw32_Inproc : FVT_lib/outp/OverrideAndLimit  SystemSampleTime=-1  VariantActivationTime=update diagram  Latency=0  AutoFrameSizeCalculation=off
      link override Signal_Limit/_maxval: Value=KOUTP_RRWheelTmpHighDTC_raw32_maxval
      link override Signal_Limit/_minval: Value=KOUTP_RRWheelTmpHighDTC_raw32_minval
      link override Signal_Override/_ovrdflg: Value=KOUTP_RRWheelTmpHighDTC_raw32_ovrdflg
      link override Signal_Override/_ovrdval: Value=KOUTP_RRWheelTmpHighDTC_raw32_ovrdval
  VDDM_RrMCUSigErrDetDTC_raw32_Inproc : FVT_lib/outp/OverrideAndLimit  SystemSampleTime=-1  VariantActivationTime=update diagram  Latency=0  AutoFrameSizeCalculation=off
      link override Signal_Limit/_maxval: Value=KOUTP_RrMCUSigErrDetDTC_raw32_maxval
      link override Signal_Limit/_minval: Value=KOUTP_RrMCUSigErrDetDTC_raw32_minval
      link override Signal_Override/_ovrdflg: Value=KOUTP_RrMCUSigErrDetDTC_raw32_ovrdflg
      link override Signal_Override/_ovrdval: Value=KOUTP_RrMCUSigErrDetDTC_raw32_ovrdval
  VDDM_RrMCUTqErrDTC_raw32_Inproc : FVT_lib/outp/OverrideAndLimit  SystemSampleTime=-1  VariantActivationTime=update diagram  Latency=0  AutoFrameSizeCalculation=off
      link override Signal_Limit/_maxval: Value=KOUTP_RrMCUTqErrDTC_raw32_maxval
      link override Signal_Limit/_minval: Value=KOUTP_RrMCUTqErrDTC_raw32_minval
      link override Signal_Override/_ovrdflg: Value=KOUTP_RrMCUTqErrDTC_raw32_ovrdflg
      link override Signal_Override/_ovrdval: Value=KOUTP_RrMCUTqErrDTC_raw32_ovrdval
  VDDM_Shifter1CSErrDTC_raw32_Inproc : FVT_lib/outp/OverrideAndLimit  SystemSampleTime=-1  VariantActivationTime=update diagram  Latency=0  AutoFrameSizeCalculation=off
      link override Signal_Limit/_maxval: Value=KOUTP_Shifter1CSErrDTC_raw32_maxval
      link override Signal_Limit/_minval: Value=KOUTP_Shifter1CSErrDTC_raw32_minval
      link override Signal_Override/_ovrdflg: Value=KOUTP_Shifter1CSErrDTC_raw32_ovrdflg
      link override Signal_Override/_ovrdval: Value=KOUTP_Shifter1CSErrDTC_raw32_ovrdval
  VDDM_Shifter1NoComDTC_raw32_Inproc : FVT_lib/outp/OverrideAndLimit  SystemSampleTime=-1  VariantActivationTime=update diagram  Latency=0  AutoFrameSizeCalculation=off
      link override Signal_Limit/_maxval: Value=KOUTP_Shifter1NoComDTC_raw32_maxval
      link override Signal_Limit/_minval: Value=KOUTP_Shifter1NoComDTC_raw32_minval
      link override Signal_Override/_ovrdflg: Value=KOUTP_Shifter1NoComDTC_raw32_ovrdflg
      link override Signal_Override/_ovrdval: Value=KOUTP_Shifter1NoComDTC_raw32_ovrdval
  VDDM_Shifter1RCErrDTC_raw32_Inproc : FVT_lib/outp/OverrideAndLimit  SystemSampleTime=-1  VariantActivationTime=update diagram  Latency=0  AutoFrameSizeCalculation=off
      link override Signal_Limit/_maxval: Value=KOUTP_Shifter1RCErrDTC_raw32_maxval
      link override Signal_Limit/_minval: Value=KOUTP_Shifter1RCErrDTC_raw32_minval
      link override Signal_Override/_ovrdflg: Value=KOUTP_Shifter1RCErrDTC_raw32_ovrdflg
      link override Signal_Override/_ovrdval: Value=KOUTP_Shifter1RCErrDTC_raw32_ovrdval
  VDDM_THCMAPTCWarning_raw32_Inproc : FVT_lib/outp/OverrideAndLimit  SystemSampleTime=-1  VariantActivationTime=update diagram  Latency=0  AutoFrameSizeCalculation=off
      link override Signal_Limit/_maxval: Value=KOUTP_THCMAPTCWarning_raw32_maxval
      link override Signal_Limit/_minval: Value=KOUTP_THCMAPTCWarning_raw32_minval
      link override Signal_Override/_ovrdflg: Value=KOUTP_THCMAPTCWarning_raw32_ovrdflg
      link override Signal_Override/_ovrdval: Value=KOUTP_THCMAPTCWarning_raw32_ovrdval
  VDDM_TailgaSWDTC_raw32_Inproc : FVT_lib/outp/OverrideAndLimit  SystemSampleTime=-1  VariantActivationTime=update diagram  Latency=0  AutoFrameSizeCalculation=off
      link override Signal_Limit/_maxval: Value=KOUTP_TailgaSWDTC_raw32_maxval
      link override Signal_Limit/_minval: Value=KOUTP_TailgaSWDTC_raw32_minval
      link override Signal_Override/_ovrdflg: Value=KOUTP_TailgaSWDTC_raw32_ovrdflg
      link override Signal_Override/_ovrdval: Value=KOUTP_TailgaSWDTC_raw32_ovrdval
  VDDM_VehMalfunLevel_enum_Inproc : FVT_lib/outp/OverrideAndLimit  SystemSampleTime=-1  VariantActivationTime=update diagram  Latency=0  AutoFrameSizeCalculation=off
      link override Signal_Limit/_maxval: Value=KOUTP_VehMalfunLevel_enum_maxval
      link override Signal_Limit/_minval: Value=KOUTP_VehMalfunLevel_enum_minval
      link override Signal_Override/_ovrdflg: Value=KOUTP_VehMalfunLevel_enum_ovrdflg
      link override Signal_Override/_ovrdval: Value=KOUTP_VehMalfunLevel_enum_ovrdval
  VDDM_ZoneSCPNoComDTC_raw32_Inproc : FVT_lib/outp/OverrideAndLimit  SystemSampleTime=-1  VariantActivationTime=update diagram  Latency=0  AutoFrameSizeCalculation=off
      link override Signal_Limit/_maxval: Value=KOUTP_ZoneSCPNoComDTC_raw32_maxval
      link override Signal_Limit/_minval: Value=KOUTP_ZoneSCPNoComDTC_raw32_minval
      link override Signal_Override/_ovrdflg: Value=KOUTP_ZoneSCPNoComDTC_raw32_ovrdflg
      link override Signal_Override/_ovrdval: Value=KOUTP_ZoneSCPNoComDTC_raw32_ovrdval
  VDHP_ActAPSPosn_pct_Inproc : FVT_lib/outp/OverrideAndLimit  SystemSampleTime=-1  VariantActivationTime=update diagram  Latency=0  AutoFrameSizeCalculation=off
      link override Signal_Limit/_maxval: Value=KOUTP_ActAPSPosn_pct_maxval
      link override Signal_Limit/_minval: Value=KOUTP_ActAPSPosn_pct_minval
      link override Signal_Override/_ovrdflg: Value=KOUTP_ActAPSPosn_pct_ovrdflg
      link override Signal_Override/_ovrdval: Value=KOUTP_ActAPSPosn_pct_ovrdval
  VDHP_EAPS1MIN_pct_Inproc : FVT_lib/outp/OverrideAndLimit  SystemSampleTime=-1  VariantActivationTime=update diagram  Latency=0  AutoFrameSizeCalculation=off
      link override Signal_Limit/_maxval: Value=KOUTP_EAPS1MIN_pct_maxval
      link override Signal_Limit/_minval: Value=KOUTP_EAPS1MIN_pct_minval
      link override Signal_Override/_ovrdflg: Value=KOUTP_EAPS1MIN_pct_ovrdflg
      link override Signal_Override/_ovrdval: Value=KOUTP_EAPS1MIN_pct_ovrdval
  VDHP_EAPS2MIN_pct_Inproc : FVT_lib/outp/OverrideAndLimit  SystemSampleTime=-1  VariantActivationTime=update diagram  Latency=0  AutoFrameSizeCalculation=off
      link override Signal_Limit/_maxval: Value=KOUTP_EAPS2MIN_pct_maxval
      link override Signal_Limit/_minval: Value=KOUTP_EAPS2MIN_pct_minval
      link override Signal_Override/_ovrdflg: Value=KOUTP_EAPS2MIN_pct_ovrdflg
      link override Signal_Override/_ovrdval: Value=KOUTP_EAPS2MIN_pct_ovrdval
  VDKC_DKCAuthSta_enum_Inproc : FVT_lib/outp/OverrideAndLimit  SystemSampleTime=-1  VariantActivationTime=update diagram  Latency=0  AutoFrameSizeCalculation=off
      link override Signal_Limit/_maxval: Value=KOUTP_DKCAuthSta_enum_maxval
      link override Signal_Limit/_minval: Value=KOUTP_DKCAuthSta_enum_minval
      link override Signal_Override/_ovrdflg: Value=KOUTP_DKCAuthSta_enum_ovrdflg
      link override Signal_Override/_ovrdval: Value=KOUTP_DKCAuthSta_enum_ovrdval
  VDKC_DKCTimeSN_cnt_Inproc : FVT_lib/outp/OverrideAndLimit  SystemSampleTime=-1  VariantActivationTime=update diagram  Latency=0  AutoFrameSizeCalculation=off
      link override Signal_Limit/_maxval: Value=KOUTP_DKCTimeSN_cnt_maxval
      link override Signal_Limit/_minval: Value=KOUTP_DKCTimeSN_cnt_minval
      link override Signal_Override/_ovrdflg: Value=KOUTP_DKCTimeSN_cnt_ovrdflg
      link override Signal_Override/_ovrdval: Value=KOUTP_DKCTimeSN_cnt_ovrdval
  VNMM_ActiveWU_flg_Inproc : FVT_lib/outp/OverrideAndLimit  SystemSampleTime=-1  VariantActivationTime=update diagram  Latency=0  AutoFrameSizeCalculation=off
      link override Signal_Limit/_maxval: Value=KOUTP_ActiveWU_flg_maxval
      link override Signal_Limit/_minval: Value=KOUTP_ActiveWU_flg_minval
      link override Signal_Override/_ovrdflg: Value=KOUTP_ActiveWU_flg_ovrdflg
      link override Signal_Override/_ovrdval: Value=KOUTP_ActiveWU_flg_ovrdval
  VNMM_AllCANTxReq_flg_Inproc : FVT_lib/outp/OverrideAndLimit  SystemSampleTime=-1  VariantActivationTime=update diagram  Latency=0  AutoFrameSizeCalculation=off
      link override Signal_Limit/_maxval: Value=KOUTP_AllCANTxReq_flg_maxval
      link override Signal_Limit/_minval: Value=KOUTP_AllCANTxReq_flg_minval
      link override Signal_Override/_ovrdflg: Value=KOUTP_AllCANTxReq_flg_ovrdflg
      link override Signal_Override/_ovrdval: Value=KOUTP_AllCANTxReq_flg_ovrdval
  VNMM_Awake_enum_Inproc : FVT_lib/outp/OverrideAndLimit  SystemSampleTime=-1  VariantActivationTime=update diagram  Latency=0  AutoFrameSizeCalculation=off
      link override Signal_Limit/_maxval: Value=KOUTP_Awake_enum_maxval
      link override Signal_Limit/_minval: Value=KOUTP_Awake_enum_minval
      link override Signal_Override/_ovrdflg: Value=KOUTP_Awake_enum_ovrdflg
      link override Signal_Override/_ovrdval: Value=KOUTP_Awake_enum_ovrdval
  VNMM_CSB_flg_Inproc : FVT_lib/outp/OverrideAndLimit  SystemSampleTime=-1  VariantActivationTime=update diagram  Latency=0  AutoFrameSizeCalculation=off
      link override Signal_Limit/_maxval: Value=KOUTP_CSB_flg_maxval
      link override Signal_Limit/_minval: Value=KOUTP_CSB_flg_minval
      link override Signal_Override/_ovrdflg: Value=KOUTP_CSB_flg_ovrdflg
      link override Signal_Override/_ovrdval: Value=KOUTP_CSB_flg_ovrdval
  VNMM_ErrorState_enum_Inproc : FVT_lib/outp/OverrideAndLimit  SystemSampleTime=-1  VariantActivationTime=update diagram  Latency=0  AutoFrameSizeCalculation=off
      link override Signal_Limit/_maxval: Value=KOUTP_ErrorState_enum_maxval
      link override Signal_Limit/_minval: Value=KOUTP_ErrorState_enum_minval
      link override Signal_Override/_ovrdflg: Value=KOUTP_ErrorState_enum_ovrdflg
      link override Signal_Override/_ovrdval: Value=KOUTP_ErrorState_enum_ovrdval
  VNMM_NMmTxReq_flg_Inproc : FVT_lib/outp/OverrideAndLimit  SystemSampleTime=-1  VariantActivationTime=update diagram  Latency=0  AutoFrameSizeCalculation=off
      link override Signal_Limit/_maxval: Value=KOUTP_NMmTxReq_flg_maxval
      link override Signal_Limit/_minval: Value=KOUTP_NMmTxReq_flg_minval
      link override Signal_Override/_ovrdflg: Value=KOUTP_NMmTxReq_flg_ovrdflg
      link override Signal_Override/_ovrdval: Value=KOUTP_NMmTxReq_flg_ovrdval
  VNMM_NetworkReq_flg_Inproc : FVT_lib/outp/OverrideAndLimit  SystemSampleTime=-1  VariantActivationTime=update diagram  Latency=0  AutoFrameSizeCalculation=off
      link override Signal_Limit/_maxval: Value=KOUTP_NetworkReq_flg_maxval
      link override Signal_Limit/_minval: Value=KOUTP_NetworkReq_flg_minval
      link override Signal_Override/_ovrdflg: Value=KOUTP_NetworkReq_flg_ovrdflg
      link override Signal_Override/_ovrdval: Value=KOUTP_NetworkReq_flg_ovrdval
  VNMM_NodeID_enum_Inproc : FVT_lib/outp/OverrideAndLimit  SystemSampleTime=-1  VariantActivationTime=update diagram  Latency=0  AutoFrameSizeCalculation=off
      link override Signal_Limit/_maxval: Value=KOUTP_NodeID_enum_maxval
      link override Signal_Limit/_minval: Value=KOUTP_NodeID_enum_minval
      link override Signal_Override/_ovrdflg: Value=KOUTP_NodeID_enum_ovrdflg
      link override Signal_Override/_ovrdval: Value=KOUTP_NodeID_enum_ovrdval
  VNMM_PNI_flg_Inproc : FVT_lib/outp/OverrideAndLimit  SystemSampleTime=-1  VariantActivationTime=update diagram  Latency=0  AutoFrameSizeCalculation=off
      link override Signal_Limit/_maxval: Value=KOUTP_PNI_flg_maxval
      link override Signal_Limit/_minval: Value=KOUTP_PNI_flg_minval
      link override Signal_Override/_ovrdflg: Value=KOUTP_PNI_flg_ovrdflg
      link override Signal_Override/_ovrdval: Value=KOUTP_PNI_flg_ovrdval
  VNMM_RptMsgReq_flg_Inproc : FVT_lib/outp/OverrideAndLimit  SystemSampleTime=-1  VariantActivationTime=update diagram  Latency=0  AutoFrameSizeCalculation=off
      link override Signal_Limit/_maxval: Value=KOUTP_RptMsgReq_flg_maxval
      link override Signal_Limit/_minval: Value=KOUTP_RptMsgReq_flg_minval
      link override Signal_Override/_ovrdflg: Value=KOUTP_RptMsgReq_flg_ovrdflg
      link override Signal_Override/_ovrdval: Value=KOUTP_RptMsgReq_flg_ovrdval
  VNMM_SysNMmSta_enum_Inproc : FVT_lib/outp/OverrideAndLimit  SystemSampleTime=-1  VariantActivationTime=update diagram  Latency=0  AutoFrameSizeCalculation=off
      link override Signal_Limit/_maxval: Value=KOUTP_SysNMmSta_enum_maxval
      link override Signal_Limit/_minval: Value=KOUTP_SysNMmSta_enum_minval
      link override Signal_Override/_ovrdflg: Value=KOUTP_SysNMmSta_enum_ovrdflg
      link override Signal_Override/_ovrdval: Value=KOUTP_SysNMmSta_enum_ovrdval
  VNMM_WakeUp_enum_Inproc : FVT_lib/outp/OverrideAndLimit  SystemSampleTime=-1  VariantActivationTime=update diagram  Latency=0  AutoFrameSizeCalculation=off
      link override Signal_Limit/_maxval: Value=KOUTP_WakeUp_enum_maxval
      link override Signal_Limit/_minval: Value=KOUTP_WakeUp_enum_minval
      link override Signal_Override/_ovrdflg: Value=KOUTP_WakeUp_enum_ovrdflg
      link override Signal_Override/_ovrdval: Value=KOUTP_WakeUp_enum_ovrdval
  VPMM_ActiveDischargeReq_flg_Inproc : FVT_lib/outp/OverrideAndLimit  SystemSampleTime=-1  VariantActivationTime=update diagram  Latency=0  AutoFrameSizeCalculation=off
      link override Signal_Limit/_maxval: Value=KOUTP_ActiveDischargeReq_flg_maxval
      link override Signal_Limit/_minval: Value=KOUTP_ActiveDischargeReq_flg_minval
      link override Signal_Override/_ovrdflg: Value=KOUTP_ActiveDischargeReq_flg_ovrdflg
      link override Signal_Override/_ovrdval: Value=KOUTP_ActiveDischargeReq_flg_ovrdval
  VPMM_CtrlDrPwrStbA2_flg_Inproc : FVT_lib/outp/OverrideAndLimit  SystemSampleTime=-1  VariantActivationTime=update diagram  Latency=0  AutoFrameSizeCalculation=off
      link override Signal_Limit/_maxval: Value=KOUTP_CtrlDrPwrStbA2_flg_maxval
      link override Signal_Limit/_minval: Value=KOUTP_CtrlDrPwrStbA2_flg_minval
      link override Signal_Override/_ovrdflg: Value=KOUTP_CtrlDrPwrStbA2_flg_ovrdflg
      link override Signal_Override/_ovrdval: Value=KOUTP_CtrlDrPwrStbA2_flg_ovrdval
  VPMM_CtrlFrBMSCCUCIR_flg_Inproc : FVT_lib/outp/OverrideAndLimit  SystemSampleTime=-1  VariantActivationTime=update diagram  Latency=0  AutoFrameSizeCalculation=off
      link override Signal_Limit/_maxval: Value=KOUTP_CtrlFrBMSCCUCIR_flg_maxval
      link override Signal_Limit/_minval: Value=KOUTP_CtrlFrBMSCCUCIR_flg_minval
      link override Signal_Override/_ovrdflg: Value=KOUTP_CtrlFrBMSCCUCIR_flg_ovrdflg
      link override Signal_Override/_ovrdval: Value=KOUTP_CtrlFrBMSCCUCIR_flg_ovrdval
  VPMM_CtrlFrEDUINVERTER_flg_Inproc : FVT_lib/outp/OverrideAndLimit  SystemSampleTime=-1  VariantActivationTime=update diagram  Latency=0  AutoFrameSizeCalculation=off
      link override Signal_Limit/_maxval: Value=KOUTP_CtrlFrEDUINVERTER_flg_maxval
      link override Signal_Limit/_minval: Value=KOUTP_CtrlFrEDUINVERTER_flg_minval
      link override Signal_Override/_ovrdflg: Value=KOUTP_CtrlFrEDUINVERTER_flg_ovrdflg
      link override Signal_Override/_ovrdval: Value=KOUTP_CtrlFrEDUINVERTER_flg_ovrdval
  VPMM_CtrlFrPwrStbA1P_flg_Inproc : FVT_lib/outp/OverrideAndLimit  SystemSampleTime=-1  VariantActivationTime=update diagram  Latency=0  AutoFrameSizeCalculation=off
      link override Signal_Limit/_maxval: Value=KOUTP_CtrlFrPwrStbA1P_flg_maxval
      link override Signal_Limit/_minval: Value=KOUTP_CtrlFrPwrStbA1P_flg_minval
      link override Signal_Override/_ovrdflg: Value=KOUTP_CtrlFrPwrStbA1P_flg_ovrdflg
      link override Signal_Override/_ovrdval: Value=KOUTP_CtrlFrPwrStbA1P_flg_ovrdval
  VPMM_CtrlFrRC1_flg_Inproc : FVT_lib/outp/OverrideAndLimit  SystemSampleTime=-1  VariantActivationTime=update diagram  Latency=0  AutoFrameSizeCalculation=off
      link override Signal_Limit/_maxval: Value=KOUTP_CtrlFrRC1_flg_maxval
      link override Signal_Limit/_minval: Value=KOUTP_CtrlFrRC1_flg_minval
      link override Signal_Override/_ovrdflg: Value=KOUTP_CtrlFrRC1_flg_ovrdflg
      link override Signal_Override/_ovrdval: Value=KOUTP_CtrlFrRC1_flg_ovrdval
  VPMM_DCDCEnaReq_flg_Inproc : FVT_lib/outp/OverrideAndLimit  SystemSampleTime=-1  VariantActivationTime=update diagram  Latency=0  AutoFrameSizeCalculation=off
      link override Signal_Limit/_maxval: Value=KOUTP_DCDCEnaReq_flg_maxval
      link override Signal_Limit/_minval: Value=KOUTP_DCDCEnaReq_flg_minval
      link override Signal_Override/_ovrdflg: Value=KOUTP_DCDCEnaReq_flg_ovrdflg
      link override Signal_Override/_ovrdval: Value=KOUTP_DCDCEnaReq_flg_ovrdval
  VPMM_DCDCVoltSetpoint_V_Inproc : FVT_lib/outp/OverrideAndLimit  SystemSampleTime=-1  VariantActivationTime=update diagram  Latency=0  AutoFrameSizeCalculation=off
      link override Signal_Limit/_maxval: Value=KOUTP_DCDCVoltSetpoint_V_maxval
      link override Signal_Limit/_minval: Value=KOUTP_DCDCVoltSetpoint_V_minval
      link override Signal_Override/_ovrdflg: Value=KOUTP_DCDCVoltSetpoint_V_ovrdflg
      link override Signal_Override/_ovrdval: Value=KOUTP_DCDCVoltSetpoint_V_ovrdval
  VPMM_DrSeatSta_enum_Inproc : FVT_lib/outp/OverrideAndLimit  SystemSampleTime=-1  VariantActivationTime=update diagram  Latency=0  AutoFrameSizeCalculation=off
      link override Signal_Limit/_maxval: Value=KOUTP_DrSeatSta_enum_maxval
      link override Signal_Limit/_minval: Value=KOUTP_DrSeatSta_enum_minval
      link override Signal_Override/_ovrdflg: Value=KOUTP_DrSeatSta_enum_ovrdflg
      link override Signal_Override/_ovrdval: Value=KOUTP_DrSeatSta_enum_ovrdval
  VPMM_DrivetrainSelect_enum_Inproc : FVT_lib/outp/OverrideAndLimit  SystemSampleTime=-1  VariantActivationTime=update diagram  Latency=0  AutoFrameSizeCalculation=off
      link override Signal_Limit/_maxval: Value=KOUTP_DrivetrainSelect_enum_maxval
      link override Signal_Limit/_minval: Value=KOUTP_DrivetrainSelect_enum_minval
      link override Signal_Override/_ovrdflg: Value=KOUTP_DrivetrainSelect_enum_ovrdflg
      link override Signal_Override/_ovrdval: Value=KOUTP_DrivetrainSelect_enum_ovrdval
  VPMM_EvccAplusPwrUpReq_flg_Inproc : FVT_lib/outp/OverrideAndLimit  SystemSampleTime=-1  VariantActivationTime=update diagram  Latency=0  AutoFrameSizeCalculation=off
      link override Signal_Limit/_maxval: Value=KOUTP_EvccAplusPwrUpReq_flg_maxval
      link override Signal_Limit/_minval: Value=KOUTP_EvccAplusPwrUpReq_flg_minval
      link override Signal_Override/_ovrdflg: Value=KOUTP_EvccAplusPwrUpReq_flg_ovrdflg
      link override Signal_Override/_ovrdval: Value=KOUTP_EvccAplusPwrUpReq_flg_ovrdval
  VPMM_FDADC12VDetAvg_mV_Inproc : FVT_lib/outp/OverrideAndLimit  SystemSampleTime=-1  VariantActivationTime=update diagram  Latency=0  AutoFrameSizeCalculation=off
      link override Signal_Limit/_maxval: Value=KOUTP_FDADC12VDetAvg_mV_maxval
      link override Signal_Limit/_minval: Value=KOUTP_FDADC12VDetAvg_mV_minval
      link override Signal_Override/_ovrdflg: Value=KOUTP_FDADC12VDetAvg_mV_ovrdflg
      link override Signal_Override/_ovrdval: Value=KOUTP_FDADC12VDetAvg_mV_ovrdval
  VPMM_FrMCUEnaReq_flg_Inproc : FVT_lib/outp/OverrideAndLimit  SystemSampleTime=-1  VariantActivationTime=update diagram  Latency=0  AutoFrameSizeCalculation=off
      link override Signal_Limit/_maxval: Value=KOUTP_FrMCUEnaReq_flg_maxval
      link override Signal_Limit/_minval: Value=KOUTP_FrMCUEnaReq_flg_minval
      link override Signal_Override/_ovrdflg: Value=KOUTP_FrMCUEnaReq_flg_ovrdflg
      link override Signal_Override/_ovrdval: Value=KOUTP_FrMCUEnaReq_flg_ovrdval
  VPMM_HVBatCnctReq_flg_Inproc : FVT_lib/outp/OverrideAndLimit  SystemSampleTime=-1  VariantActivationTime=update diagram  Latency=0  AutoFrameSizeCalculation=off
      link override Signal_Limit/_maxval: Value=KOUTP_HVBatCnctReq_flg_maxval
      link override Signal_Limit/_minval: Value=KOUTP_HVBatCnctReq_flg_minval
      link override Signal_Override/_ovrdflg: Value=KOUTP_HVBatCnctReq_flg_ovrdflg
      link override Signal_Override/_ovrdval: Value=KOUTP_HVBatCnctReq_flg_ovrdval
  VPMM_HVPwrSta_flg_Inproc : FVT_lib/outp/OverrideAndLimit  SystemSampleTime=-1  VariantActivationTime=update diagram  Latency=0  AutoFrameSizeCalculation=off
      link override Signal_Limit/_maxval: Value=KOUTP_HVPwrSta_flg_maxval
      link override Signal_Limit/_minval: Value=KOUTP_HVPwrSta_flg_minval
      link override Signal_Override/_ovrdflg: Value=KOUTP_HVPwrSta_flg_ovrdflg
      link override Signal_Override/_ovrdval: Value=KOUTP_HVPwrSta_flg_ovrdval
  VPMM_HVSysReadyToCharge_enum_Inproc : FVT_lib/outp/OverrideAndLimit  SystemSampleTime=-1  VariantActivationTime=update diagram  Latency=0  AutoFrameSizeCalculation=off
      link override Signal_Limit/_maxval: Value=KOUTP_HVSysReadyToCharge_enum_maxval
      link override Signal_Limit/_minval: Value=KOUTP_HVSysReadyToCharge_enum_minval
      link override Signal_Override/_ovrdflg: Value=KOUTP_HVSysReadyToCharge_enum_ovrdflg
      link override Signal_Override/_ovrdval: Value=KOUTP_HVSysReadyToCharge_enum_ovrdval
  VPMM_HWResetSta_enum_Inproc : FVT_lib/outp/OverrideAndLimit  SystemSampleTime=-1  VariantActivationTime=update diagram  Latency=0  AutoFrameSizeCalculation=off
      link override Signal_Limit/_maxval: Value=KOUTP_HWResetSta_enum_maxval
      link override Signal_Limit/_minval: Value=KOUTP_HWResetSta_enum_minval
      link override Signal_Override/_ovrdflg: Value=KOUTP_HWResetSta_enum_ovrdflg
      link override Signal_Override/_ovrdval: Value=KOUTP_HWResetSta_enum_ovrdval
  VPMM_IVIPwrStaONTOPopT_s_Inproc : FVT_lib/outp/OverrideAndLimit  SystemSampleTime=-1  VariantActivationTime=update diagram  Latency=0  AutoFrameSizeCalculation=off
      link override Signal_Limit/_maxval: Value=KOUTP_IVIPwrStaONTOPopT_s_maxval
      link override Signal_Limit/_minval: Value=KOUTP_IVIPwrStaONTOPopT_s_minval
      link override Signal_Override/_ovrdflg: Value=KOUTP_IVIPwrStaONTOPopT_s_ovrdflg
      link override Signal_Override/_ovrdval: Value=KOUTP_IVIPwrStaONTOPopT_s_ovrdval
  VPMM_LVBattChrgTimeCnt_s_Inproc : FVT_lib/outp/OverrideAndLimit  SystemSampleTime=-1  VariantActivationTime=update diagram  Latency=0  AutoFrameSizeCalculation=off
      link override Signal_Limit/_maxval: Value=KOUTP_LVBattChrgTimeCnt_s_maxval
      link override Signal_Limit/_minval: Value=KOUTP_LVBattChrgTimeCnt_s_minval
      link override Signal_Override/_ovrdflg: Value=KOUTP_LVBattChrgTimeCnt_s_ovrdflg
      link override Signal_Override/_ovrdval: Value=KOUTP_LVBattChrgTimeCnt_s_ovrdval
  VPMM_LVChrgHoldTtimer_s_Inproc : FVT_lib/outp/OverrideAndLimit  SystemSampleTime=-1  VariantActivationTime=update diagram  Latency=0  AutoFrameSizeCalculation=off
      link override Signal_Limit/_maxval: Value=KOUTP_LVChrgHoldTtimer_s_maxval
      link override Signal_Limit/_minval: Value=KOUTP_LVChrgHoldTtimer_s_minval
      link override Signal_Override/_ovrdflg: Value=KOUTP_LVChrgHoldTtimer_s_ovrdflg
      link override Signal_Override/_ovrdval: Value=KOUTP_LVChrgHoldTtimer_s_ovrdval
  VPMM_LVPwrSta_flg_Inproc : FVT_lib/outp/OverrideAndLimit  SystemSampleTime=-1  VariantActivationTime=update diagram  Latency=0  AutoFrameSizeCalculation=off
      link override Signal_Limit/_maxval: Value=KOUTP_LVPwrSta_flg_maxval
      link override Signal_Limit/_minval: Value=KOUTP_LVPwrSta_flg_minval
      link override Signal_Override/_ovrdflg: Value=KOUTP_LVPwrSta_flg_ovrdflg
      link override Signal_Override/_ovrdval: Value=KOUTP_LVPwrSta_flg_ovrdval
  VPMM_LVSilentChrgLv_enum_Inproc : FVT_lib/outp/OverrideAndLimit  SystemSampleTime=-1  VariantActivationTime=update diagram  Latency=0  AutoFrameSizeCalculation=off
      link override Signal_Limit/_maxval: Value=KOUTP_LVSilentChrgLv_enum_maxval
      link override Signal_Limit/_minval: Value=KOUTP_LVSilentChrgLv_enum_minval
      link override Signal_Override/_ovrdflg: Value=KOUTP_LVSilentChrgLv_enum_ovrdflg
      link override Signal_Override/_ovrdval: Value=KOUTP_LVSilentChrgLv_enum_ovrdval
  VPMM_LVSilentChrgReq_flg_Inproc : FVT_lib/outp/OverrideAndLimit  SystemSampleTime=-1  VariantActivationTime=update diagram  Latency=0  AutoFrameSizeCalculation=off
      link override Signal_Limit/_maxval: Value=KOUTP_LVSilentChrgReq_flg_maxval
      link override Signal_Limit/_minval: Value=KOUTP_LVSilentChrgReq_flg_minval
      link override Signal_Override/_ovrdflg: Value=KOUTP_LVSilentChrgReq_flg_ovrdflg
      link override Signal_Override/_ovrdval: Value=KOUTP_LVSilentChrgReq_flg_ovrdval
  VPMM_LVSilentChrgSta_enum_Inproc : FVT_lib/outp/OverrideAndLimit  SystemSampleTime=-1  VariantActivationTime=update diagram  Latency=0  AutoFrameSizeCalculation=off
      link override Signal_Limit/_maxval: Value=KOUTP_LVSilentChrgSta_enum_maxval
      link override Signal_Limit/_minval: Value=KOUTP_LVSilentChrgSta_enum_minval
      link override Signal_Override/_ovrdflg: Value=KOUTP_LVSilentChrgSta_enum_ovrdflg
      link override Signal_Override/_ovrdval: Value=KOUTP_LVSilentChrgSta_enum_ovrdval
  VPMM_LVSysErrPwrOutErr_flg_Inproc : FVT_lib/outp/OverrideAndLimit  SystemSampleTime=-1  VariantActivationTime=update diagram  Latency=0  AutoFrameSizeCalculation=off
      link override Signal_Limit/_maxval: Value=KOUTP_LVSysErrPwrOutErr_flg_maxval
      link override Signal_Limit/_minval: Value=KOUTP_LVSysErrPwrOutErr_flg_minval
      link override Signal_Override/_ovrdflg: Value=KOUTP_LVSysErrPwrOutErr_flg_ovrdflg
      link override Signal_Override/_ovrdval: Value=KOUTP_LVSysErrPwrOutErr_flg_ovrdval
  VPMM_LowSOCWarn_enum_Inproc : FVT_lib/outp/OverrideAndLimit  SystemSampleTime=-1  VariantActivationTime=update diagram  Latency=0  AutoFrameSizeCalculation=off
      link override Signal_Limit/_maxval: Value=KOUTP_LowSOCWarn_enum_maxval
      link override Signal_Limit/_minval: Value=KOUTP_LowSOCWarn_enum_minval
      link override Signal_Override/_ovrdflg: Value=KOUTP_LowSOCWarn_enum_ovrdflg
      link override Signal_Override/_ovrdval: Value=KOUTP_LowSOCWarn_enum_ovrdval
  VPMM_OTAPwrReqOFFChkSta_enum_Inproc : FVT_lib/outp/OverrideAndLimit  SystemSampleTime=-1  VariantActivationTime=update diagram  Latency=0  AutoFrameSizeCalculation=off
      link override Signal_Limit/_maxval: Value=KOUTP_OTAPwrReqOFFChkSta_enum_maxval
      link override Signal_Limit/_minval: Value=KOUTP_OTAPwrReqOFFChkSta_enum_minval
      link override Signal_Override/_ovrdflg: Value=KOUTP_OTAPwrReqOFFChkSta_enum_ovrdflg
      link override Signal_Override/_ovrdval: Value=KOUTP_OTAPwrReqOFFChkSta_enum_ovrdval
  VPMM_OTAPwrReqStdChkSta_enum_Inproc : FVT_lib/outp/OverrideAndLimit  SystemSampleTime=-1  VariantActivationTime=update diagram  Latency=0  AutoFrameSizeCalculation=off
      link override Signal_Limit/_maxval: Value=KOUTP_OTAPwrReqStdChkSta_enum_maxval
      link override Signal_Limit/_minval: Value=KOUTP_OTAPwrReqStdChkSta_enum_minval
      link override Signal_Override/_ovrdflg: Value=KOUTP_OTAPwrReqStdChkSta_enum_ovrdflg
      link override Signal_Override/_ovrdval: Value=KOUTP_OTAPwrReqStdChkSta_enum_ovrdval
  VPMM_PMMAllowECUSleep_flg_Inproc : FVT_lib/outp/OverrideAndLimit  SystemSampleTime=-1  VariantActivationTime=update diagram  Latency=0  AutoFrameSizeCalculation=off
      link override Signal_Limit/_maxval: Value=KOUTP_PMMAllowECUSleep_flg_maxval
      link override Signal_Limit/_minval: Value=KOUTP_PMMAllowECUSleep_flg_minval
      link override Signal_Override/_ovrdflg: Value=KOUTP_PMMAllowECUSleep_flg_ovrdflg
      link override Signal_Override/_ovrdval: Value=KOUTP_PMMAllowECUSleep_flg_ovrdval
  VPMM_PowerDownFault_enum_Inproc : FVT_lib/outp/OverrideAndLimit  SystemSampleTime=-1  VariantActivationTime=update diagram  Latency=0  AutoFrameSizeCalculation=off
      link override Signal_Limit/_maxval: Value=KOUTP_PowerDownFault_enum_maxval
      link override Signal_Limit/_minval: Value=KOUTP_PowerDownFault_enum_minval
      link override Signal_Override/_ovrdflg: Value=KOUTP_PowerDownFault_enum_ovrdflg
      link override Signal_Override/_ovrdval: Value=KOUTP_PowerDownFault_enum_ovrdval
  VPMM_PowerDownState_enum_Inproc : FVT_lib/outp/OverrideAndLimit  SystemSampleTime=-1  VariantActivationTime=update diagram  Latency=0  AutoFrameSizeCalculation=off
      link override Signal_Limit/_maxval: Value=KOUTP_PowerDownState_enum_maxval
      link override Signal_Limit/_minval: Value=KOUTP_PowerDownState_enum_minval
      link override Signal_Override/_ovrdflg: Value=KOUTP_PowerDownState_enum_ovrdflg
      link override Signal_Override/_ovrdval: Value=KOUTP_PowerDownState_enum_ovrdval
  VPMM_PowerSta_enum_Inproc : FVT_lib/outp/OverrideAndLimit  SystemSampleTime=-1  VariantActivationTime=update diagram  Latency=0  AutoFrameSizeCalculation=off
      link override Signal_Limit/_maxval: Value=KOUTP_PowerSta_enum_maxval
      link override Signal_Limit/_minval: Value=KOUTP_PowerSta_enum_minval
      link override Signal_Override/_ovrdflg: Value=KOUTP_PowerSta_enum_ovrdflg
      link override Signal_Override/_ovrdval: Value=KOUTP_PowerSta_enum_ovrdval
  VPMM_PowerUpFault_enum_Inproc : FVT_lib/outp/OverrideAndLimit  SystemSampleTime=-1  VariantActivationTime=update diagram  Latency=0  AutoFrameSizeCalculation=off
      link override Signal_Limit/_maxval: Value=KOUTP_PowerUpFault_enum_maxval
      link override Signal_Limit/_minval: Value=KOUTP_PowerUpFault_enum_minval
      link override Signal_Override/_ovrdflg: Value=KOUTP_PowerUpFault_enum_ovrdflg
      link override Signal_Override/_ovrdval: Value=KOUTP_PowerUpFault_enum_ovrdval
  VPMM_PowerUpState_enum_Inproc : FVT_lib/outp/OverrideAndLimit  SystemSampleTime=-1  VariantActivationTime=update diagram  Latency=0  AutoFrameSizeCalculation=off
      link override Signal_Limit/_maxval: Value=KOUTP_PowerUpState_enum_maxval
      link override Signal_Limit/_minval: Value=KOUTP_PowerUpState_enum_minval
      link override Signal_Override/_ovrdflg: Value=KOUTP_PowerUpState_enum_ovrdflg
      link override Signal_Override/_ovrdval: Value=KOUTP_PowerUpState_enum_ovrdval
  VPMM_PwrDownReq_enum_Inproc : FVT_lib/outp/OverrideAndLimit  SystemSampleTime=-1  VariantActivationTime=update diagram  Latency=0  AutoFrameSizeCalculation=off
      link override Signal_Limit/_maxval: Value=KOUTP_PwrDownReq_enum_maxval
      link override Signal_Limit/_minval: Value=KOUTP_PwrDownReq_enum_minval
      link override Signal_Override/_ovrdflg: Value=KOUTP_PwrDownReq_enum_ovrdflg
      link override Signal_Override/_ovrdval: Value=KOUTP_PwrDownReq_enum_ovrdval
  VPMM_PwrReq_OTA_enum_Inproc : FVT_lib/outp/OverrideAndLimit  SystemSampleTime=-1  VariantActivationTime=update diagram  Latency=0  AutoFrameSizeCalculation=off
      link override Signal_Limit/_maxval: Value=KOUTP_PwrReq_OTA_enum_maxval
      link override Signal_Limit/_minval: Value=KOUTP_PwrReq_OTA_enum_minval
      link override Signal_Override/_ovrdflg: Value=KOUTP_PwrReq_OTA_enum_ovrdflg
      link override Signal_Override/_ovrdval: Value=KOUTP_PwrReq_OTA_enum_ovrdval
  VPMM_PwrStaConstraint_enum_Inproc : FVT_lib/outp/OverrideAndLimit  SystemSampleTime=-1  VariantActivationTime=update diagram  Latency=0  AutoFrameSizeCalculation=off
      link override Signal_Limit/_maxval: Value=KOUTP_PwrStaConstraint_enum_maxval
      link override Signal_Limit/_minval: Value=KOUTP_PwrStaConstraint_enum_minval
      link override Signal_Override/_ovrdflg: Value=KOUTP_PwrStaConstraint_enum_ovrdflg
      link override Signal_Override/_ovrdval: Value=KOUTP_PwrStaConstraint_enum_ovrdval
  VPMM_PwrStaONTOPopReq_flg_Inproc : FVT_lib/outp/OverrideAndLimit  SystemSampleTime=-1  VariantActivationTime=update diagram  Latency=0  AutoFrameSizeCalculation=off
      link override Signal_Limit/_maxval: Value=KOUTP_PwrStaONTOPopReq_flg_maxval
      link override Signal_Limit/_minval: Value=KOUTP_PwrStaONTOPopReq_flg_minval
      link override Signal_Override/_ovrdflg: Value=KOUTP_PwrStaONTOPopReq_flg_ovrdflg
      link override Signal_Override/_ovrdval: Value=KOUTP_PwrStaONTOPopReq_flg_ovrdval
  VPMM_PwrStaSelect_enum_Inproc : FVT_lib/outp/OverrideAndLimit  SystemSampleTime=-1  VariantActivationTime=update diagram  Latency=0  AutoFrameSizeCalculation=off
      link override Signal_Limit/_maxval: Value=KOUTP_PwrStaSelect_enum_maxval
      link override Signal_Limit/_minval: Value=KOUTP_PwrStaSelect_enum_minval
      link override Signal_Override/_ovrdflg: Value=KOUTP_PwrStaSelect_enum_ovrdflg
      link override Signal_Override/_ovrdval: Value=KOUTP_PwrStaSelect_enum_ovrdval
  VPMM_PwrStaTOSta_enum_Inproc : FVT_lib/outp/OverrideAndLimit  SystemSampleTime=-1  VariantActivationTime=update diagram  Latency=0  AutoFrameSizeCalculation=off
      link override Signal_Limit/_maxval: Value=KOUTP_PwrStaTOSta_enum_maxval
      link override Signal_Limit/_minval: Value=KOUTP_PwrStaTOSta_enum_minval
      link override Signal_Override/_ovrdflg: Value=KOUTP_PwrStaTOSta_enum_ovrdflg
      link override Signal_Override/_ovrdval: Value=KOUTP_PwrStaTOSta_enum_ovrdval
  VPMM_PwrUpReq_enum_Inproc : FVT_lib/outp/OverrideAndLimit  SystemSampleTime=-1  VariantActivationTime=update diagram  Latency=0  AutoFrameSizeCalculation=off
      link override Signal_Limit/_maxval: Value=KOUTP_PwrUpReq_enum_maxval
      link override Signal_Limit/_minval: Value=KOUTP_PwrUpReq_enum_minval
      link override Signal_Override/_ovrdflg: Value=KOUTP_PwrUpReq_enum_ovrdflg
      link override Signal_Override/_ovrdval: Value=KOUTP_PwrUpReq_enum_ovrdval
  VPMM_ReVehThdChkSta_enum_Inproc : FVT_lib/outp/OverrideAndLimit  SystemSampleTime=-1  VariantActivationTime=update diagram  Latency=0  AutoFrameSizeCalculation=off
      link override Signal_Limit/_maxval: Value=KOUTP_ReVehThdChkSta_enum_maxval
      link override Signal_Limit/_minval: Value=KOUTP_ReVehThdChkSta_enum_minval
      link override Signal_Override/_ovrdflg: Value=KOUTP_ReVehThdChkSta_enum_ovrdflg
      link override Signal_Override/_ovrdval: Value=KOUTP_ReVehThdChkSta_enum_ovrdval
  VPMM_RrMCUEnaReq_flg_Inproc : FVT_lib/outp/OverrideAndLimit  SystemSampleTime=-1  VariantActivationTime=update diagram  Latency=0  AutoFrameSizeCalculation=off
      link override Signal_Limit/_maxval: Value=KOUTP_RrMCUEnaReq_flg_maxval
      link override Signal_Limit/_minval: Value=KOUTP_RrMCUEnaReq_flg_minval
      link override Signal_Override/_ovrdflg: Value=KOUTP_RrMCUEnaReq_flg_ovrdflg
      link override Signal_Override/_ovrdval: Value=KOUTP_RrMCUEnaReq_flg_ovrdval
  VPMM_Sched_ChgTOSta_enum_Inproc : FVT_lib/outp/OverrideAndLimit  SystemSampleTime=-1  VariantActivationTime=update diagram  Latency=0  AutoFrameSizeCalculation=off
      link override Signal_Limit/_maxval: Value=KOUTP_Sched_ChgTOSta_enum_maxval
      link override Signal_Limit/_minval: Value=KOUTP_Sched_ChgTOSta_enum_minval
      link override Signal_Override/_ovrdflg: Value=KOUTP_Sched_ChgTOSta_enum_ovrdflg
      link override Signal_Override/_ovrdval: Value=KOUTP_Sched_ChgTOSta_enum_ovrdval
  VPMM_SilentChkAllowSleep_flg_Inproc : FVT_lib/outp/OverrideAndLimit  SystemSampleTime=-1  VariantActivationTime=update diagram  Latency=0  AutoFrameSizeCalculation=off
      link override Signal_Limit/_maxval: Value=KOUTP_SilentChkAllowSleep_flg_maxval
      link override Signal_Limit/_minval: Value=KOUTP_SilentChkAllowSleep_flg_minval
      link override Signal_Override/_ovrdflg: Value=KOUTP_SilentChkAllowSleep_flg_ovrdflg
      link override Signal_Override/_ovrdval: Value=KOUTP_SilentChkAllowSleep_flg_ovrdval
  VPMM_SysPowerMode_enum_Inproc : FVT_lib/outp/OverrideAndLimit  SystemSampleTime=-1  VariantActivationTime=update diagram  Latency=0  AutoFrameSizeCalculation=off
      link override Signal_Limit/_maxval: Value=KOUTP_SysPowerMode_enum_maxval
      link override Signal_Limit/_minval: Value=KOUTP_SysPowerMode_enum_minval
      link override Signal_Override/_ovrdflg: Value=KOUTP_SysPowerMode_enum_ovrdflg
      link override Signal_Override/_ovrdval: Value=KOUTP_SysPowerMode_enum_ovrdval
  VPMM_TCountSta_enum_Inproc : FVT_lib/outp/OverrideAndLimit  SystemSampleTime=-1  VariantActivationTime=update diagram  Latency=0  AutoFrameSizeCalculation=off
      link override Signal_Limit/_maxval: Value=KOUTP_TCountSta_enum_maxval
      link override Signal_Limit/_minval: Value=KOUTP_TCountSta_enum_minval
      link override Signal_Override/_ovrdflg: Value=KOUTP_TCountSta_enum_ovrdflg
      link override Signal_Override/_ovrdval: Value=KOUTP_TCountSta_enum_ovrdval
  VPMM_TimerAllowSleep_flg_Inproc : FVT_lib/outp/OverrideAndLimit  SystemSampleTime=-1  VariantActivationTime=update diagram  Latency=0  AutoFrameSizeCalculation=off
      link override Signal_Limit/_maxval: Value=KOUTP_TimerAllowSleep_flg_maxval
      link override Signal_Limit/_minval: Value=KOUTP_TimerAllowSleep_flg_minval
      link override Signal_Override/_ovrdflg: Value=KOUTP_TimerAllowSleep_flg_ovrdflg
      link override Signal_Override/_ovrdval: Value=KOUTP_TimerAllowSleep_flg_ovrdval
  VSYS_AcoreRebootCmdACK_flg_Inproc : FVT_lib/outp/OverrideAndLimit  SystemSampleTime=-1  VariantActivationTime=update diagram  Latency=0  AutoFrameSizeCalculation=off
      link override Signal_Limit/_maxval: Value=KOUTP_AcoreRebootCmdACK_flg_maxval
      link override Signal_Limit/_minval: Value=KOUTP_AcoreRebootCmdACK_flg_minval
      link override Signal_Override/_ovrdflg: Value=KOUTP_AcoreRebootCmdACK_flg_ovrdflg
      link override Signal_Override/_ovrdval: Value=KOUTP_AcoreRebootCmdACK_flg_ovrdval
  VSYS_CarModel1_cnt_Inproc : FVT_lib/outp/OverrideAndLimit  SystemSampleTime=-1  VariantActivationTime=update diagram  Latency=0  AutoFrameSizeCalculation=off
      link override Signal_Limit/_maxval: Value=KOUTP_CarModel1_cnt_maxval
      link override Signal_Limit/_minval: Value=KOUTP_CarModel1_cnt_minval
      link override Signal_Override/_ovrdflg: Value=KOUTP_CarModel1_cnt_ovrdflg
      link override Signal_Override/_ovrdval: Value=KOUTP_CarModel1_cnt_ovrdval
  VSYS_CarModel2_cnt_Inproc : FVT_lib/outp/OverrideAndLimit  SystemSampleTime=-1  VariantActivationTime=update diagram  Latency=0  AutoFrameSizeCalculation=off
      link override Signal_Limit/_maxval: Value=KOUTP_CarModel2_cnt_maxval
      link override Signal_Limit/_minval: Value=KOUTP_CarModel2_cnt_minval
      link override Signal_Override/_ovrdflg: Value=KOUTP_CarModel2_cnt_ovrdflg
      link override Signal_Override/_ovrdval: Value=KOUTP_CarModel2_cnt_ovrdval
  VSYS_CarModel3_cnt_Inproc : FVT_lib/outp/OverrideAndLimit  SystemSampleTime=-1  VariantActivationTime=update diagram  Latency=0  AutoFrameSizeCalculation=off
      link override Signal_Limit/_maxval: Value=KOUTP_CarModel3_cnt_maxval
      link override Signal_Limit/_minval: Value=KOUTP_CarModel3_cnt_minval
      link override Signal_Override/_ovrdflg: Value=KOUTP_CarModel3_cnt_ovrdflg
      link override Signal_Override/_ovrdval: Value=KOUTP_CarModel3_cnt_ovrdval
  VSYS_Change1_cnt_Inproc : FVT_lib/outp/OverrideAndLimit  SystemSampleTime=-1  VariantActivationTime=update diagram  Latency=0  AutoFrameSizeCalculation=off
      link override Signal_Limit/_maxval: Value=KOUTP_Change1_cnt_maxval
      link override Signal_Limit/_minval: Value=KOUTP_Change1_cnt_minval
      link override Signal_Override/_ovrdflg: Value=KOUTP_Change1_cnt_ovrdflg
      link override Signal_Override/_ovrdval: Value=KOUTP_Change1_cnt_ovrdval
  VSYS_Change2_cnt_Inproc : FVT_lib/outp/OverrideAndLimit  SystemSampleTime=-1  VariantActivationTime=update diagram  Latency=0  AutoFrameSizeCalculation=off
      link override Signal_Limit/_maxval: Value=KOUTP_Change2_cnt_maxval
      link override Signal_Limit/_minval: Value=KOUTP_Change2_cnt_minval
      link override Signal_Override/_ovrdflg: Value=KOUTP_Change2_cnt_ovrdflg
      link override Signal_Override/_ovrdval: Value=KOUTP_Change2_cnt_ovrdval
  VSYS_Country1_cnt_Inproc : FVT_lib/outp/OverrideAndLimit  SystemSampleTime=-1  VariantActivationTime=update diagram  Latency=0  AutoFrameSizeCalculation=off
      link override Signal_Limit/_maxval: Value=KOUTP_Country1_cnt_maxval
      link override Signal_Limit/_minval: Value=KOUTP_Country1_cnt_minval
      link override Signal_Override/_ovrdflg: Value=KOUTP_Country1_cnt_ovrdflg
      link override Signal_Override/_ovrdval: Value=KOUTP_Country1_cnt_ovrdval
  VSYS_Country2_cnt_Inproc : FVT_lib/outp/OverrideAndLimit  SystemSampleTime=-1  VariantActivationTime=update diagram  Latency=0  AutoFrameSizeCalculation=off
      link override Signal_Limit/_maxval: Value=KOUTP_Country2_cnt_maxval
      link override Signal_Limit/_minval: Value=KOUTP_Country2_cnt_minval
      link override Signal_Override/_ovrdflg: Value=KOUTP_Country2_cnt_ovrdflg
      link override Signal_Override/_ovrdval: Value=KOUTP_Country2_cnt_ovrdval
  VSYS_CurrentNmState_enum_Inproc : FVT_lib/outp/OverrideAndLimit  SystemSampleTime=-1  VariantActivationTime=update diagram  Latency=0  AutoFrameSizeCalculation=off
      link override Signal_Limit/_maxval: Value=KOUTP_CurrentNmState_enum_maxval
      link override Signal_Limit/_minval: Value=KOUTP_CurrentNmState_enum_minval
      link override Signal_Override/_ovrdflg: Value=KOUTP_CurrentNmState_enum_ovrdflg
      link override Signal_Override/_ovrdval: Value=KOUTP_CurrentNmState_enum_ovrdval
  VSYS_Dash1_cnt_Inproc : FVT_lib/outp/OverrideAndLimit  SystemSampleTime=-1  VariantActivationTime=update diagram  Latency=0  AutoFrameSizeCalculation=off
      link override Signal_Limit/_maxval: Value=KOUTP_Dash1_cnt_maxval
      link override Signal_Limit/_minval: Value=KOUTP_Dash1_cnt_minval
      link override Signal_Override/_ovrdflg: Value=KOUTP_Dash1_cnt_ovrdflg
      link override Signal_Override/_ovrdval: Value=KOUTP_Dash1_cnt_ovrdval
  VSYS_Dash2_cnt_Inproc : FVT_lib/outp/OverrideAndLimit  SystemSampleTime=-1  VariantActivationTime=update diagram  Latency=0  AutoFrameSizeCalculation=off
      link override Signal_Limit/_maxval: Value=KOUTP_Dash2_cnt_maxval
      link override Signal_Limit/_minval: Value=KOUTP_Dash2_cnt_minval
      link override Signal_Override/_ovrdflg: Value=KOUTP_Dash2_cnt_ovrdflg
      link override Signal_Override/_ovrdval: Value=KOUTP_Dash2_cnt_ovrdval
  VSYS_ECU1_cnt_Inproc : FVT_lib/outp/OverrideAndLimit  SystemSampleTime=-1  VariantActivationTime=update diagram  Latency=0  AutoFrameSizeCalculation=off
      link override Signal_Limit/_maxval: Value=KOUTP_ECU1_cnt_maxval
      link override Signal_Limit/_minval: Value=KOUTP_ECU1_cnt_minval
      link override Signal_Override/_ovrdflg: Value=KOUTP_ECU1_cnt_ovrdflg
      link override Signal_Override/_ovrdval: Value=KOUTP_ECU1_cnt_ovrdval
  VSYS_ECU2_cnt_Inproc : FVT_lib/outp/OverrideAndLimit  SystemSampleTime=-1  VariantActivationTime=update diagram  Latency=0  AutoFrameSizeCalculation=off
      link override Signal_Limit/_maxval: Value=KOUTP_ECU2_cnt_maxval
      link override Signal_Limit/_minval: Value=KOUTP_ECU2_cnt_minval
      link override Signal_Override/_ovrdflg: Value=KOUTP_ECU2_cnt_ovrdflg
      link override Signal_Override/_ovrdval: Value=KOUTP_ECU2_cnt_ovrdval
  VSYS_FdcSlpReqRisingEdge_flg_Inproc : FVT_lib/outp/OverrideAndLimit  SystemSampleTime=-1  VariantActivationTime=update diagram  Latency=0  AutoFrameSizeCalculation=off
      link override Signal_Limit/_maxval: Value=KOUTP_FdcSlpReqRisingEdge_flg_maxval
      link override Signal_Limit/_minval: Value=KOUTP_FdcSlpReqRisingEdge_flg_minval
      link override Signal_Override/_ovrdflg: Value=KOUTP_FdcSlpReqRisingEdge_flg_ovrdflg
      link override Signal_Override/_ovrdval: Value=KOUTP_FdcSlpReqRisingEdge_flg_ovrdval
  VSYS_FdcSlpTime_sec_Inproc : FVT_lib/outp/OverrideAndLimit  SystemSampleTime=-1  VariantActivationTime=update diagram  Latency=0  AutoFrameSizeCalculation=off
      link override Signal_Limit/_maxval: Value=KOUTP_FdcSlpTime_sec_maxval
      link override Signal_Limit/_minval: Value=KOUTP_FdcSlpTime_sec_minval
      link override Signal_Override/_ovrdflg: Value=KOUTP_FdcSlpTime_sec_ovrdflg
      link override Signal_Override/_ovrdval: Value=KOUTP_FdcSlpTime_sec_ovrdval
  VSYS_HWVer1_cnt_Inproc : FVT_lib/outp/OverrideAndLimit  SystemSampleTime=-1  VariantActivationTime=update diagram  Latency=0  AutoFrameSizeCalculation=off
      link override Signal_Limit/_maxval: Value=KOUTP_HWVer1_cnt_maxval
      link override Signal_Limit/_minval: Value=KOUTP_HWVer1_cnt_minval
      link override Signal_Override/_ovrdflg: Value=KOUTP_HWVer1_cnt_ovrdflg
      link override Signal_Override/_ovrdval: Value=KOUTP_HWVer1_cnt_ovrdval
  VSYS_HWVer2_cnt_Inproc : FVT_lib/outp/OverrideAndLimit  SystemSampleTime=-1  VariantActivationTime=update diagram  Latency=0  AutoFrameSizeCalculation=off
      link override Signal_Limit/_maxval: Value=KOUTP_HWVer2_cnt_maxval
      link override Signal_Limit/_minval: Value=KOUTP_HWVer2_cnt_minval
      link override Signal_Override/_ovrdflg: Value=KOUTP_HWVer2_cnt_ovrdflg
      link override Signal_Override/_ovrdval: Value=KOUTP_HWVer2_cnt_ovrdval
  VSYS_HWVer3_cnt_Inproc : FVT_lib/outp/OverrideAndLimit  SystemSampleTime=-1  VariantActivationTime=update diagram  Latency=0  AutoFrameSizeCalculation=off
      link override Signal_Limit/_maxval: Value=KOUTP_HWVer3_cnt_maxval
      link override Signal_Limit/_minval: Value=KOUTP_HWVer3_cnt_minval
      link override Signal_Override/_ovrdflg: Value=KOUTP_HWVer3_cnt_ovrdflg
      link override Signal_Override/_ovrdval: Value=KOUTP_HWVer3_cnt_ovrdval
  VSYS_Major1_cnt_Inproc : FVT_lib/outp/OverrideAndLimit  SystemSampleTime=-1  VariantActivationTime=update diagram  Latency=0  AutoFrameSizeCalculation=off
      link override Signal_Limit/_maxval: Value=KOUTP_Major1_cnt_maxval
      link override Signal_Limit/_minval: Value=KOUTP_Major1_cnt_minval
      link override Signal_Override/_ovrdflg: Value=KOUTP_Major1_cnt_ovrdflg
      link override Signal_Override/_ovrdval: Value=KOUTP_Major1_cnt_ovrdval
  VSYS_Major2_cnt_Inproc : FVT_lib/outp/OverrideAndLimit  SystemSampleTime=-1  VariantActivationTime=update diagram  Latency=0  AutoFrameSizeCalculation=off
      link override Signal_Limit/_maxval: Value=KOUTP_Major2_cnt_maxval
      link override Signal_Limit/_minval: Value=KOUTP_Major2_cnt_minval
      link override Signal_Override/_ovrdflg: Value=KOUTP_Major2_cnt_ovrdflg
      link override Signal_Override/_ovrdval: Value=KOUTP_Major2_cnt_ovrdval
  VSYS_Minor1_cnt_Inproc : FVT_lib/outp/OverrideAndLimit  SystemSampleTime=-1  VariantActivationTime=update diagram  Latency=0  AutoFrameSizeCalculation=off
      link override Signal_Limit/_maxval: Value=KOUTP_Minor1_cnt_maxval
      link override Signal_Limit/_minval: Value=KOUTP_Minor1_cnt_minval
      link override Signal_Override/_ovrdflg: Value=KOUTP_Minor1_cnt_ovrdflg
      link override Signal_Override/_ovrdval: Value=KOUTP_Minor1_cnt_ovrdval
  VSYS_Minor2_cnt_Inproc : FVT_lib/outp/OverrideAndLimit  SystemSampleTime=-1  VariantActivationTime=update diagram  Latency=0  AutoFrameSizeCalculation=off
      link override Signal_Limit/_maxval: Value=KOUTP_Minor2_cnt_maxval
      link override Signal_Limit/_minval: Value=KOUTP_Minor2_cnt_minval
      link override Signal_Override/_ovrdflg: Value=KOUTP_Minor2_cnt_ovrdflg
      link override Signal_Override/_ovrdval: Value=KOUTP_Minor2_cnt_ovrdval
  VSYS_NvWriteReqRisingEdge_flg_Inproc : FVT_lib/outp/OverrideAndLimit  SystemSampleTime=-1  VariantActivationTime=update diagram  Latency=0  AutoFrameSizeCalculation=off
      link override Signal_Limit/_maxval: Value=KOUTP_NvWriteReqRisingEdge_flg_maxval
      link override Signal_Limit/_minval: Value=KOUTP_NvWriteReqRisingEdge_flg_minval
      link override Signal_Override/_ovrdflg: Value=KOUTP_NvWriteReqRisingEdge_flg_ovrdflg
      link override Signal_Override/_ovrdval: Value=KOUTP_NvWriteReqRisingEdge_flg_ovrdval
  VSYS_Patch1_cnt_Inproc : FVT_lib/outp/OverrideAndLimit  SystemSampleTime=-1  VariantActivationTime=update diagram  Latency=0  AutoFrameSizeCalculation=off
      link override Signal_Limit/_maxval: Value=KOUTP_Patch1_cnt_maxval
      link override Signal_Limit/_minval: Value=KOUTP_Patch1_cnt_minval
      link override Signal_Override/_ovrdflg: Value=KOUTP_Patch1_cnt_ovrdflg
      link override Signal_Override/_ovrdval: Value=KOUTP_Patch1_cnt_ovrdval
  VSYS_Patch2_cnt_Inproc : FVT_lib/outp/OverrideAndLimit  SystemSampleTime=-1  VariantActivationTime=update diagram  Latency=0  AutoFrameSizeCalculation=off
      link override Signal_Limit/_maxval: Value=KOUTP_Patch2_cnt_maxval
      link override Signal_Limit/_minval: Value=KOUTP_Patch2_cnt_minval
      link override Signal_Override/_ovrdflg: Value=KOUTP_Patch2_cnt_ovrdflg
      link override Signal_Override/_ovrdval: Value=KOUTP_Patch2_cnt_ovrdval
  VSYS_PmicBootReason_enum_Inproc : FVT_lib/outp/OverrideAndLimit  SystemSampleTime=-1  VariantActivationTime=update diagram  Latency=0  AutoFrameSizeCalculation=off
      link override Signal_Limit/_maxval: Value=KOUTP_PmicBootReason_enum_maxval
      link override Signal_Limit/_minval: Value=KOUTP_PmicBootReason_enum_minval
      link override Signal_Override/_ovrdflg: Value=KOUTP_PmicBootReason_enum_ovrdflg
      link override Signal_Override/_ovrdval: Value=KOUTP_PmicBootReason_enum_ovrdval
  VSYS_SHA1_cnt_Inproc : FVT_lib/outp/OverrideAndLimit  SystemSampleTime=-1  VariantActivationTime=update diagram  Latency=0  AutoFrameSizeCalculation=off
      link override Signal_Limit/_maxval: Value=KOUTP_SHA1_cnt_maxval
      link override Signal_Limit/_minval: Value=KOUTP_SHA1_cnt_minval
      link override Signal_Override/_ovrdflg: Value=KOUTP_SHA1_cnt_ovrdflg
      link override Signal_Override/_ovrdval: Value=KOUTP_SHA1_cnt_ovrdval
  VSYS_SHA2_cnt_Inproc : FVT_lib/outp/OverrideAndLimit  SystemSampleTime=-1  VariantActivationTime=update diagram  Latency=0  AutoFrameSizeCalculation=off
      link override Signal_Limit/_maxval: Value=KOUTP_SHA2_cnt_maxval
      link override Signal_Limit/_minval: Value=KOUTP_SHA2_cnt_minval
      link override Signal_Override/_ovrdflg: Value=KOUTP_SHA2_cnt_ovrdflg
      link override Signal_Override/_ovrdval: Value=KOUTP_SHA2_cnt_ovrdval
  VSYS_SHA3_cnt_Inproc : FVT_lib/outp/OverrideAndLimit  SystemSampleTime=-1  VariantActivationTime=update diagram  Latency=0  AutoFrameSizeCalculation=off
      link override Signal_Limit/_maxval: Value=KOUTP_SHA3_cnt_maxval
      link override Signal_Limit/_minval: Value=KOUTP_SHA3_cnt_minval
      link override Signal_Override/_ovrdflg: Value=KOUTP_SHA3_cnt_ovrdflg
      link override Signal_Override/_ovrdval: Value=KOUTP_SHA3_cnt_ovrdval
  VSYS_SHA4_cnt_Inproc : FVT_lib/outp/OverrideAndLimit  SystemSampleTime=-1  VariantActivationTime=update diagram  Latency=0  AutoFrameSizeCalculation=off
      link override Signal_Limit/_maxval: Value=KOUTP_SHA4_cnt_maxval
      link override Signal_Limit/_minval: Value=KOUTP_SHA4_cnt_minval
      link override Signal_Override/_ovrdflg: Value=KOUTP_SHA4_cnt_ovrdflg
      link override Signal_Override/_ovrdval: Value=KOUTP_SHA4_cnt_ovrdval
  VSYS_SHA5_cnt_Inproc : FVT_lib/outp/OverrideAndLimit  SystemSampleTime=-1  VariantActivationTime=update diagram  Latency=0  AutoFrameSizeCalculation=off
      link override Signal_Limit/_maxval: Value=KOUTP_SHA5_cnt_maxval
      link override Signal_Limit/_minval: Value=KOUTP_SHA5_cnt_minval
      link override Signal_Override/_ovrdflg: Value=KOUTP_SHA5_cnt_ovrdflg
      link override Signal_Override/_ovrdval: Value=KOUTP_SHA5_cnt_ovrdval
  VSYS_SHA6_cnt_Inproc : FVT_lib/outp/OverrideAndLimit  SystemSampleTime=-1  VariantActivationTime=update diagram  Latency=0  AutoFrameSizeCalculation=off
      link override Signal_Limit/_maxval: Value=KOUTP_SHA6_cnt_maxval
      link override Signal_Limit/_minval: Value=KOUTP_SHA6_cnt_minval
      link override Signal_Override/_ovrdflg: Value=KOUTP_SHA6_cnt_ovrdflg
      link override Signal_Override/_ovrdval: Value=KOUTP_SHA6_cnt_ovrdval
  VSYS_SHA7_cnt_Inproc : FVT_lib/outp/OverrideAndLimit  SystemSampleTime=-1  VariantActivationTime=update diagram  Latency=0  AutoFrameSizeCalculation=off
      link override Signal_Limit/_maxval: Value=KOUTP_SHA7_cnt_maxval
      link override Signal_Limit/_minval: Value=KOUTP_SHA7_cnt_minval
      link override Signal_Override/_ovrdflg: Value=KOUTP_SHA7_cnt_ovrdflg
      link override Signal_Override/_ovrdval: Value=KOUTP_SHA7_cnt_ovrdval
  VSYS_SHA8_cnt_Inproc : FVT_lib/outp/OverrideAndLimit  SystemSampleTime=-1  VariantActivationTime=update diagram  Latency=0  AutoFrameSizeCalculation=off
      link override Signal_Limit/_maxval: Value=KOUTP_SHA8_cnt_maxval
      link override Signal_Limit/_minval: Value=KOUTP_SHA8_cnt_minval
      link override Signal_Override/_ovrdflg: Value=KOUTP_SHA8_cnt_ovrdflg
      link override Signal_Override/_ovrdval: Value=KOUTP_SHA8_cnt_ovrdval
  VSYS_Variation_cnt_Inproc : FVT_lib/outp/OverrideAndLimit  SystemSampleTime=-1  VariantActivationTime=update diagram  Latency=0  AutoFrameSizeCalculation=off
      link override Signal_Limit/_maxval: Value=KOUTP_Variation_cnt_maxval
      link override Signal_Limit/_minval: Value=KOUTP_Variation_cnt_minval
      link override Signal_Override/_ovrdflg: Value=KOUTP_Variation_cnt_ovrdflg
      link override Signal_Override/_ovrdval: Value=KOUTP_Variation_cnt_ovrdval
  VSYS_WisrBootReason_raw32_Inproc : FVT_lib/outp/OverrideAndLimit  SystemSampleTime=-1  VariantActivationTime=update diagram  Latency=0  AutoFrameSizeCalculation=off
      link override Signal_Limit/_maxval: Value=KOUTP_WisrBootReason_raw32_maxval
      link override Signal_Limit/_minval: Value=KOUTP_WisrBootReason_raw32_minval
      link override Signal_Override/_ovrdflg: Value=KOUTP_WisrBootReason_raw32_ovrdflg
      link override Signal_Override/_ovrdval: Value=KOUTP_WisrBootReason_raw32_ovrdval
  VTHC_ACForceOFF_flg_Inproc : FVT_lib/outp/OverrideAndLimit  SystemSampleTime=-1  VariantActivationTime=update diagram  Latency=0  AutoFrameSizeCalculation=off
      link override Signal_Limit/_maxval: Value=KOUTP_ACForceOFF_flg_maxval
      link override Signal_Limit/_minval: Value=KOUTP_ACForceOFF_flg_minval
      link override Signal_Override/_ovrdflg: Value=KOUTP_ACForceOFF_flg_ovrdflg
      link override Signal_Override/_ovrdval: Value=KOUTP_ACForceOFF_flg_ovrdval
  VTHC_ACModeMem_enum_Inproc : FVT_lib/outp/OverrideAndLimit  SystemSampleTime=-1  VariantActivationTime=update diagram  Latency=0  AutoFrameSizeCalculation=off
      link override Signal_Limit/_maxval: Value=KOUTP_ACModeMem_enum_maxval
      link override Signal_Limit/_minval: Value=KOUTP_ACModeMem_enum_minval
      link override Signal_Override/_ovrdflg: Value=KOUTP_ACModeMem_enum_ovrdflg
      link override Signal_Override/_ovrdval: Value=KOUTP_ACModeMem_enum_ovrdval
  VTHC_ACSubMode_enum_Inproc : FVT_lib/outp/OverrideAndLimit  SystemSampleTime=-1  VariantActivationTime=update diagram  Latency=0  AutoFrameSizeCalculation=off
      link override Signal_Limit/_maxval: Value=KOUTP_ACSubMode_enum_maxval
      link override Signal_Limit/_minval: Value=KOUTP_ACSubMode_enum_minval
      link override Signal_Override/_ovrdflg: Value=KOUTP_ACSubMode_enum_ovrdflg
      link override Signal_Override/_ovrdval: Value=KOUTP_ACSubMode_enum_ovrdval
  VTHC_AirIntenZone1M_enum_Inproc : FVT_lib/outp/OverrideAndLimit  SystemSampleTime=-1  VariantActivationTime=update diagram  Latency=0  AutoFrameSizeCalculation=off
      link override Signal_Limit/_maxval: Value=KOUTP_AirIntenZone1M_enum_maxval
      link override Signal_Limit/_minval: Value=KOUTP_AirIntenZone1M_enum_minval
      link override Signal_Override/_ovrdflg: Value=KOUTP_AirIntenZone1M_enum_ovrdflg
      link override Signal_Override/_ovrdval: Value=KOUTP_AirIntenZone1M_enum_ovrdval
  VTHC_BatteryMode_enum_Inproc : FVT_lib/outp/OverrideAndLimit  SystemSampleTime=-1  VariantActivationTime=update diagram  Latency=0  AutoFrameSizeCalculation=off
      link override Signal_Limit/_maxval: Value=KOUTP_BatteryMode_enum_maxval
      link override Signal_Limit/_minval: Value=KOUTP_BatteryMode_enum_minval
      link override Signal_Override/_ovrdflg: Value=KOUTP_BatteryMode_enum_ovrdflg
      link override Signal_Override/_ovrdval: Value=KOUTP_BatteryMode_enum_ovrdval
  VTHC_CCUACLampSts_flg_Inproc : FVT_lib/outp/OverrideAndLimit  SystemSampleTime=-1  VariantActivationTime=update diagram  Latency=0  AutoFrameSizeCalculation=off
      link override Signal_Limit/_maxval: Value=KOUTP_CCUACLampSts_flg_maxval
      link override Signal_Limit/_minval: Value=KOUTP_CCUACLampSts_flg_minval
      link override Signal_Override/_ovrdflg: Value=KOUTP_CCUACLampSts_flg_ovrdflg
      link override Signal_Override/_ovrdval: Value=KOUTP_CCUACLampSts_flg_ovrdval
  VTHC_CCUACMaxLampSts_flg_Inproc : FVT_lib/outp/OverrideAndLimit  SystemSampleTime=-1  VariantActivationTime=update diagram  Latency=0  AutoFrameSizeCalculation=off
      link override Signal_Limit/_maxval: Value=KOUTP_CCUACMaxLampSts_flg_maxval
      link override Signal_Limit/_minval: Value=KOUTP_CCUACMaxLampSts_flg_minval
      link override Signal_Override/_ovrdflg: Value=KOUTP_CCUACMaxLampSts_flg_ovrdflg
      link override Signal_Override/_ovrdval: Value=KOUTP_CCUACMaxLampSts_flg_ovrdval
  VTHC_CCUAutoLampSts_flg_Inproc : FVT_lib/outp/OverrideAndLimit  SystemSampleTime=-1  VariantActivationTime=update diagram  Latency=0  AutoFrameSizeCalculation=off
